simulink model "MHILSimHWImpl"  (R2024a)
settings: Solver=FixedStepDiscrete  StartTime=0.0  StopTime=2e-4  FixedStep=4e-9  RelTol=1e-3
values from neighbouring files (symbols this model uses):
  cfg = tddbl_model    [HILSimModel.m]
undefined symbols (not defined in the file or in its folder): AXI4, dt, hw, ip, Lite, xc7z020clg400
libraries: hdlBasic x1497, hdlUtilities x3, vmcUtilities x1
(part 2 of 11)

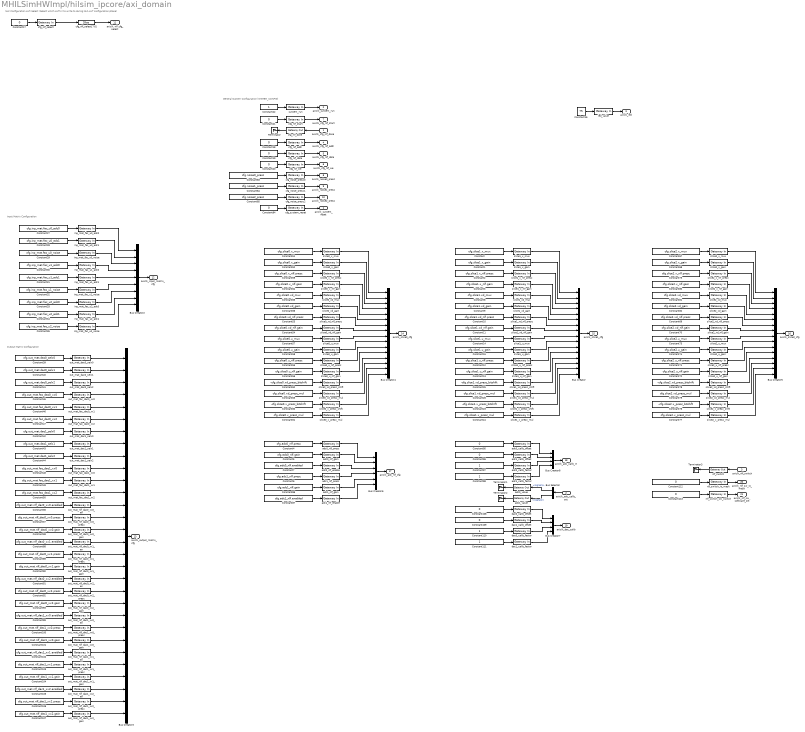
== system MHILSimHWImpl/hilsim_ipcore/axi_domain ==
  note: Input Matrix Configuration
  note: General System Configuration (SYSTEM_CONFIG)
  note: NLF Configuration LUT-Select (Select which LUT(s) to write to during NLF-LUT configuration phase)
  note: Output Matrix Configuration
  axiclk_cfg_nlf_done : Inport
  axiclk_adc_calib_out : Inport  Port=2
  axiclk_nlf_switch : Inport  Port=3
  Bus Creator : BusCreator  Inputs=16
  Bus Creator2 : BusCreator  Inputs=9
  Bus Creator3 : BusCreator  Inputs=30
  Bus Creator4 : BusCreator  Inputs=16
  Bus Creator5 : BusCreator  Inputs=16
  Bus Creator6 : BusCreator  Inputs=6
  Bus Creator7 : BusCreator  Inputs=4
  Bus Creator8 : BusCreator  Inputs=4
  Bus Selector : BusSelector  OutputSignals=signal1,signal2
  Constant : Constant  Value=cfg.slice1.x_mux
  Constant1 : Constant  Value=cfg.slice1.x_gain
  Constant10 : Constant  Value=cfg.slice1.xd_nlf.presc
  Constant100 : Constant  Value=cfg.out_mat.nlf_dac1_xx0.presc
  Constant101 : Constant  Value=cfg.out_mat.nlf_dac1_xx0.gain
  Constant102 : Constant  Value=cfg.out_mat.nlf_dac1_xx1.enabled
  Constant103 : Constant  Value=cfg.out_mat.nlf_dac1_xx1.presc
  Constant104 : Constant  Value=cfg.out_mat.nlf_dac1_xx1.gain
  Constant105 : Constant  Value=cfg.out_mat.nlf_dac1_xx2.enabled
  Constant106 : Constant  Value=cfg.out_mat.nlf_dac1_xx2.presc
  Constant107 : Constant  Value=cfg.out_mat.nlf_dac1_xx2.gain
  Constant{95,108,112..113} (4 alike) : Constant  Value=0  VectorParams1D=off
  Constant{17..21,94,96,109} (8 alike) : Constant  Value=0
  Constant11 : Constant  Value=cfg.slice1.xd_nlf.gain
  Constant{97..98,110..111} (4 alike) : Constant  VectorParams1D=off
  Constant12 : Constant  Value=cfg.slice1.u_nlf.presc
  Constant13 : Constant  Value=cfg.slice1.u_nlf.gain
  Constant14 : Constant  Value=cfg.slice1.u_mux
  Constant15 : Constant  Value=cfg.slice1.u_gain
  Constant16 : Constant  Value=75
  Constant2 : Constant  Value=cfg.slice1.x_nlf.presc
  Constant22 : Constant
  Constant23 : Constant  Value=-cfg.slice1.x_presc_bitshift  VectorParams1D=off
  Constant24 : Constant  Value=cfg.slice1.x_presc_mul
  Constant25 : Constant  Value=-cfg.slice1.xd_presc_bitshift
  Constant26 : Constant  Value=cfg.slice1.xd_presc_mul
  Constant27 : Constant  Value=cfg.inp_mat.fac_u0_adc0
  Constant28 : Constant  Value=cfg.inp_mat.fac_u0_adc1
  Constant29 : Constant  Value=cfg.inp_mat.fac_u0_noise
  Constant3 : Constant  Value=cfg.slice1.x_nlf.gain
  Constant30 : Constant  Value=cfg.inp_mat.fac_u1_adc0
  Constant31 : Constant  Value=cfg.inp_mat.fac_u1_adc1
  Constant32 : Constant  Value=cfg.inp_mat.fac_u1_noise
  Constant33 : Constant  Value=cfg.inp_mat.fac_u2_adc0
  Constant34 : Constant  Value=cfg.inp_mat.fac_u2_adc1
  Constant35 : Constant  Value=cfg.inp_mat.fac_u2_noise
  Constant36 : Constant  Value=cfg.out_mat.nlf_dac0_xx0.enabled
  Constant37 : Constant  Value=cfg.out_mat.nlf_dac0_xx0.presc
  Constant38 : Constant  Value=cfg.out_mat.nlf_dac0_xx0.gain
  Constant39 : Constant  Value=cfg.out_mat.dac0_selx0
  Constant4 : Constant  Value=cfg.adc0_nlf.presc
  Constant40 : Constant  Value=cfg.out_mat.dac0_selx1
  Constant41 : Constant  Value=cfg.out_mat.dac0_selx2
  Constant42 : Constant  Value=cfg.out_mat.dac1_selx0
  Constant43 : Constant  Value=cfg.out_mat.dac1_selx1
  Constant44 : Constant  Value=cfg.out_mat.dac1_selx2
  Constant45 : Constant  Value=cfg.out_mat.fac_dac0_xx0
  Constant46 : Constant  Value=cfg.out_mat.fac_dac0_xx1
  Constant47 : Constant  Value=cfg.out_mat.fac_dac0_xx2
  Constant48 : Constant  Value=cfg.out_mat.fac_dac1_xx0
  Constant49 : Constant  Value=cfg.out_mat.fac_dac1_xx1
  Constant5 : Constant  Value=cfg.adc0_nlf.gain
  Constant50 : Constant  Value=cfg.out_mat.fac_dac1_xx2
  Constant51 : Constant  Value=cfg.slice0.x_mux
  Constant52 : Constant  Value=cfg.slice0.x_gain
  Constant53 : Constant  Value=cfg.slice0.xd_nlf.presc
  Constant54 : Constant  Value=cfg.slice0.xd_nlf.gain
  Constant55 : Constant  Value=cfg.slice0.u_nlf.presc
  Constant56 : Constant  Value=cfg.slice0.u_nlf.gain
  Constant57 : Constant  Value=cfg.slice0.u_mux
  Constant58 : Constant  Value=cfg.slice0.u_gain
  Constant59 : Constant  Value=cfg.slice0.x_nlf.presc
  Constant6 : Constant  Value=cfg.adc1_nlf.presc
  Constant60 : Constant  Value=-cfg.slice0.x_presc_bitshift  VectorParams1D=off
  Constant61 : Constant  Value=cfg.slice0.x_presc_mul
  Constant62 : Constant  Value=-cfg.slice0.xd_presc_bitshift
  Constant63 : Constant  Value=cfg.slice0.xd_presc_mul
  Constant64 : Constant  Value=cfg.slice0.x_nlf.gain
  Constant65 : Constant  Value=cfg.slice0.xd_mux
  Constant66 : Constant  Value=cfg.slice0.xd_gain
  Constant67 : Constant  Value=cfg.slice2.x_mux
  Constant68 : Constant  Value=cfg.slice2.x_gain
  Constant69 : Constant  Value=cfg.slice2.xd_nlf.presc
  Constant7 : Constant  Value=cfg.adc0_nlf.enabled
  Constant70 : Constant  Value=cfg.slice2.xd_nlf.gain
  Constant71 : Constant  Value=cfg.slice2.u_nlf.presc
  Constant72 : Constant  Value=cfg.slice2.u_nlf.gain
  Constant73 : Constant  Value=cfg.slice2.u_mux
  Constant74 : Constant  Value=cfg.slice2.u_gain
  Constant75 : Constant  Value=cfg.slice2.x_nlf.presc
  Constant76 : Constant  Value=-cfg.slice2.x_presc_bitshift  VectorParams1D=off
  Constant77 : Constant  Value=cfg.slice2.x_presc_mul
  Constant78 : Constant  Value=-cfg.slice2.xd_presc_bitshift
  Constant79 : Constant  Value=cfg.slice2.xd_presc_mul
  Constant8 : Constant  Value=cfg.slice1.xd_mux
  Constant80 : Constant  Value=cfg.slice2.x_nlf.gain
  Constant81 : Constant  Value=cfg.slice2.xd_mux
  Constant82 : Constant  Value=cfg.slice2.xd_gain
  Constant83 : Constant  Value=cfg.noise0_presc
  Constant84 : Constant  Value=cfg.noise1_presc
  Constant85 : Constant  Value=cfg.noise2_presc
  Constant86 : Constant  Value=cfg.adc1_nlf.gain
  Constant87 : Constant  Value=cfg.adc1_nlf.enabled
  Constant88 : Constant  Value=cfg.out_mat.nlf_dac0_xx1.enabled
  Constant89 : Constant  Value=cfg.out_mat.nlf_dac0_xx1.presc
  Constant9 : Constant  Value=cfg.slice1.xd_gain
  Constant90 : Constant  Value=cfg.out_mat.nlf_dac0_xx1.gain
  Constant91 : Constant  Value=cfg.out_mat.nlf_dac0_xx2.enabled
  Constant92 : Constant  Value=cfg.out_mat.nlf_dac0_xx2.presc
  Constant93 : Constant  Value=cfg.out_mat.nlf_dac0_xx2.gain
  Constant99 : Constant  Value=cfg.out_mat.nlf_dac1_xx0.enabled
  Terminator{,1..3} (4 alike) : Terminator
  adc0_calib_factor : hdlBasic/Gateway In  gui_display_data_type=Fixed-point  arith_type=Signed (2's comp)  n_bits=dt.const.sz  bin_pt=dt.const.bin  preci_type=Single  exp_width=8  frac_width=24  rows=1  columns=1  quantization=Truncate  overflow=Wrap  period=hw.t_axi  UseAsADC=off  ADCChannel='1'  interface=AXI4-Lite  automatic_assignment=off  address_offset=ip.offsets.calib + hex2dec('08')  intf_name='axi_b'  intf_description=''  default_value=0  timing_constraint=None  locs_specified=off  LOCs={}  io_standard={}  inherit_from_input=off  hdl_port=on  XmcBlockStatus=1  maskContainerNames=group4  block_type=gatewayin  block_config=sysgen:gateway_in_config  block_width_w=590  block_height_w=620  block_width=640  block_height=850
  adc0_calib_offset : hdlBasic/Gateway In  gui_display_data_type=Fixed-point  arith_type=Signed (2's comp)  n_bits=dt.slice.sz  bin_pt=dt.slice.bin  preci_type=Single  exp_width=8  frac_width=24  rows=1  columns=1  quantization=Truncate  overflow=Wrap  period=hw.t_axi  UseAsADC=off  ADCChannel='1'  interface=AXI4-Lite  automatic_assignment=off  address_offset=ip.offsets.calib + hex2dec('00')  intf_name='axi_b'  intf_description=''  default_value=0  timing_constraint=None  locs_specified=off  LOCs={}  io_standard={}  inherit_from_input=off  hdl_port=on  XmcBlockStatus=1  maskContainerNames=group4  block_type=gatewayin  block_config=sysgen:gateway_in_config  block_width_w=590  block_height_w=620  block_width=640  block_height=850
  adc0_nlf_enable : hdlBasic/Gateway In  gui_display_data_type=Boolean  arith_type=Boolean  n_bits=8  bin_pt=0  preci_type=Single  exp_width=8  frac_width=24  rows=1  columns=1  quantization=Truncate  overflow=Wrap  period=hw.t_axi  UseAsADC=off  ADCChannel='1'  interface=AXI4-Lite  automatic_assignment=off  address_offset=ip.offsets.adc_nlf_cfg + hex2dec('08')  intf_name=''  intf_description=''  default_value=0  timing_constraint=None  locs_specified=off  LOCs={}  io_standard={}  inherit_from_input=off  hdl_port=on  XmcBlockStatus=1  maskContainerNames=group4  block_type=gatewayin  block_config=sysgen:gateway_in_config  block_width_w=590  block_height_w=620  block_width=640  block_height=850
  adc0_nlf_gain : hdlBasic/Gateway In  gui_display_data_type=Fixed-point  arith_type=Signed (2's comp)  n_bits=dt.const.sz  bin_pt=dt.const.bin  preci_type=Single  exp_width=8  frac_width=24  rows=1  columns=1  quantization=Truncate  overflow=Wrap  period=hw.t_axi  UseAsADC=off  ADCChannel='1'  interface=AXI4-Lite  automatic_assignment=off  address_offset=ip.offsets.adc_nlf_cfg + hex2dec('04')  intf_name=''  intf_description=''  default_value=0  timing_constraint=None  locs_specified=off  LOCs={}  io_standard={}  inherit_from_input=off  hdl_port=on  XmcBlockStatus=1  maskContainerNames=group4  block_type=gatewayin  block_config=sysgen:gateway_in_config  block_width_w=590  block_height_w=620  block_width=640  block_height=850
  adc0_nlf_presc : hdlBasic/Gateway In  gui_display_data_type=Fixed-point  arith_type=Signed (2's comp)  n_bits=dt.const.sz  bin_pt=dt.const.bin  preci_type=Single  exp_width=8  frac_width=24  rows=1  columns=1  quantization=Truncate  overflow=Wrap  period=hw.t_axi  UseAsADC=off  ADCChannel='1'  interface=AXI4-Lite  automatic_assignment=off  address_offset=ip.offsets.adc_nlf_cfg + hex2dec('00')  intf_name=''  intf_description=''  default_value=0  timing_constraint=None  locs_specified=off  LOCs={}  io_standard={}  inherit_from_input=off  hdl_port=on  XmcBlockStatus=1  maskContainerNames=group4  block_type=gatewayin  block_config=sysgen:gateway_in_config  block_width_w=590  block_height_w=620  block_width=640  block_height=850
  adc0_value : hdlBasic/Gateway Out  inherit_from_input=off  hdl_port=on  rows=1  columns=1  UseAsDAC=off  DACChannel='1'  interface=AXI4-Lite  automatic_assignment=off  address_offset=ip.offsets.calib + hex2dec('10')  intf_name='axi_b'  intf_description=''  timing_constraint=None  locs_specified=off  LOCs={}  io_standard={}  XmcBlockStatus=1  maskContainerNames=group4  block_type=gatewayout  block_config=sysgen:gateway_out_config  block_width_w=590  block_height_w=620  block_width=620  block_height=750
  adc1_calib_factor : hdlBasic/Gateway In  gui_display_data_type=Fixed-point  arith_type=Signed (2's comp)  n_bits=dt.const.sz  bin_pt=dt.const.bin  preci_type=Single  exp_width=8  frac_width=24  rows=1  columns=1  quantization=Truncate  overflow=Wrap  period=hw.t_axi  UseAsADC=off  ADCChannel='1'  interface=AXI4-Lite  automatic_assignment=off  address_offset=ip.offsets.calib + hex2dec('0c')  intf_name='axi_b'  intf_description=''  default_value=0  timing_constraint=None  locs_specified=off  LOCs={}  io_standard={}  inherit_from_input=off  hdl_port=on  XmcBlockStatus=1  maskContainerNames=group4  block_type=gatewayin  block_config=sysgen:gateway_in_config  block_width_w=590  block_height_w=620  block_width=640  block_height=850
  adc1_calib_offset : hdlBasic/Gateway In  gui_display_data_type=Fixed-point  arith_type=Signed (2's comp)  n_bits=dt.slice.sz  bin_pt=dt.slice.bin  preci_type=Single  exp_width=8  frac_width=24  rows=1  columns=1  quantization=Truncate  overflow=Wrap  period=hw.t_axi  UseAsADC=off  ADCChannel='1'  interface=AXI4-Lite  automatic_assignment=off  address_offset=ip.offsets.calib + hex2dec('04')  intf_name='axi_b'  intf_description=''  default_value=0  timing_constraint=None  locs_specified=off  LOCs={}  io_standard={}  inherit_from_input=off  hdl_port=on  XmcBlockStatus=1  maskContainerNames=group4  block_type=gatewayin  block_config=sysgen:gateway_in_config  block_width_w=590  block_height_w=620  block_width=640  block_height=850
  adc1_nlf_enable : hdlBasic/Gateway In  gui_display_data_type=Boolean  arith_type=Boolean  n_bits=8  bin_pt=0  preci_type=Single  exp_width=8  frac_width=24  rows=1  columns=1  quantization=Truncate  overflow=Wrap  period=hw.t_axi  UseAsADC=off  ADCChannel='1'  interface=AXI4-Lite  automatic_assignment=off  address_offset=ip.offsets.adc_nlf_cfg + hex2dec('14')  intf_name=''  intf_description=''  default_value=0  timing_constraint=None  locs_specified=off  LOCs={}  io_standard={}  inherit_from_input=off  hdl_port=on  XmcBlockStatus=1  maskContainerNames=group4  block_type=gatewayin  block_config=sysgen:gateway_in_config  block_width_w=590  block_height_w=620  block_width=640  block_height=850
  adc1_nlf_gain : hdlBasic/Gateway In  gui_display_data_type=Fixed-point  arith_type=Signed (2's comp)  n_bits=dt.const.sz  bin_pt=dt.const.bin  preci_type=Single  exp_width=8  frac_width=24  rows=1  columns=1  quantization=Truncate  overflow=Wrap  period=hw.t_axi  UseAsADC=off  ADCChannel='1'  interface=AXI4-Lite  automatic_assignment=off  address_offset=ip.offsets.adc_nlf_cfg + hex2dec('10')  intf_name=''  intf_description=''  default_value=0  timing_constraint=None  locs_specified=off  LOCs={}  io_standard={}  inherit_from_input=off  hdl_port=on  XmcBlockStatus=1  maskContainerNames=group4  block_type=gatewayin  block_config=sysgen:gateway_in_config  block_width_w=590  block_height_w=620  block_width=640  block_height=850
  adc1_nlf_presc : hdlBasic/Gateway In  gui_display_data_type=Fixed-point  arith_type=Signed (2's comp)  n_bits=dt.const.sz  bin_pt=dt.const.bin  preci_type=Single  exp_width=8  frac_width=24  rows=1  columns=1  quantization=Truncate  overflow=Wrap  period=hw.t_axi  UseAsADC=off  ADCChannel='1'  interface=AXI4-Lite  automatic_assignment=off  address_offset=ip.offsets.adc_nlf_cfg + hex2dec('0c')  intf_name=''  intf_description=''  default_value=0  timing_constraint=None  locs_specified=off  LOCs={}  io_standard={}  inherit_from_input=off  hdl_port=on  XmcBlockStatus=1  maskContainerNames=group4  block_type=gatewayin  block_config=sysgen:gateway_in_config  block_width_w=590  block_height_w=620  block_width=640  block_height=850
  adc1_value : hdlBasic/Gateway Out  inherit_from_input=off  hdl_port=on  rows=1  columns=1  UseAsDAC=off  DACChannel='1'  interface=AXI4-Lite  automatic_assignment=off  address_offset=ip.offsets.calib + hex2dec('14')  intf_name='axi_b'  intf_description=''  timing_constraint=None  locs_specified=off  LOCs={}  io_standard={}  XmcBlockStatus=1  maskContainerNames=group4  block_type=gatewayout  block_config=sysgen:gateway_out_config  block_width_w=590  block_height_w=620  block_width=620  block_height=750
  cfg_nlf_addr : hdlBasic/Gateway In  gui_display_data_type=Fixed-point  arith_type=Unsigned  n_bits=ip.f_nlf.lut_addr_bits  bin_pt=0  preci_type=Single  exp_width=8  frac_width=24  rows=1  columns=1  quantization=Truncate  overflow=Wrap  period=hw.t_axi  UseAsADC=off  ADCChannel='1'  interface=AXI4-Lite  automatic_assignment=off  address_offset=ip.offsets.system_cfg + hex2dec('14')  intf_name=''  intf_description=''  default_value=0  timing_constraint=None  locs_specified=off  LOCs={}  io_standard={}  inherit_from_input=off  hdl_port=on  XmcBlockStatus=1  maskContainerNames=group4  block_type=gatewayin  block_config=sysgen:gateway_in_config  block_width_w=590  block_height_w=620  block_width=640  block_height=850
  cfg_nlf_data : hdlBasic/Gateway In  gui_display_data_type=Fixed-point  arith_type=Signed (2's comp)  n_bits=dt.nlf.sz  bin_pt=dt.nlf.bin  preci_type=Single  exp_width=8  frac_width=24  rows=1  columns=1  quantization=Truncate  overflow=Wrap  period=hw.t_axi  UseAsADC=off  ADCChannel='1'  interface=AXI4-Lite  automatic_assignment=off  address_offset=ip.offsets.system_cfg + hex2dec('18')  intf_name=''  intf_description=''  default_value=0  timing_constraint=None  locs_specified=off  LOCs={}  io_standard={}  inherit_from_input=off  hdl_port=on  XmcBlockStatus=1  maskContainerNames=group4  block_type=gatewayin  block_config=sysgen:gateway_in_config  block_width_w=590  block_height_w=620  block_width=640  block_height=850
  cfg_nlf_done : hdlBasic/Gateway Out  inherit_from_input=off  hdl_port=on  rows=1  columns=1  UseAsDAC=off  DACChannel='1'  interface=AXI4-Lite  automatic_assignment=off  address_offset=ip.offsets.system_cfg + hex2dec('08')  intf_name=''  intf_description=''  timing_constraint=None  locs_specified=off  LOCs={}  io_standard={}  XmcBlockStatus=1  maskContainerNames=group4  block_type=gatewayout  block_config=sysgen:gateway_out_config  block_width_w=590  block_height_w=620  block_width=620  block_height=750
  cfg_nlf_select : hdlBasic/Gateway In  gui_display_data_type=Fixed-point  arith_type=Unsigned  n_bits=32  bin_pt=0  preci_type=Single  exp_width=8  frac_width=24  rows=1  columns=1  quantization=Truncate  overflow=Wrap  period=hw.t_axi  UseAsADC=off  ADCChannel='1'  interface=AXI4-Lite  automatic_assignment=off  address_offset=ip.offsets.system_cfg + hex2dec('10')  intf_name=''  intf_description=''  default_value=0  timing_constraint=None  locs_specified=off  LOCs={}  io_standard={}  inherit_from_input=off  hdl_port=on  XmcBlockStatus=1  maskContainerNames=group4  block_type=gatewayin  block_config=sysgen:gateway_in_config  block_width_w=590  block_height_w=620  block_width=640  block_height=850
  cfg_nlf_select[7:0] : hdlBasic/Slice  nbits=8  boolean_output=off  mode=Lower Bit Location + Width  bit1=0  base1=MSB of Input  bit0=0  base0=LSB of Input  XmcBlockStatus=1  maskContainerNames=group1  block_type=slice  block_config=sysgen:Slice_config
  cfg_nlf_start : hdlBasic/Gateway In  gui_display_data_type=Boolean  arith_type=Boolean  n_bits=dt.nlf.sz  bin_pt=dt.nlf.bin  preci_type=Single  exp_width=8  frac_width=24  rows=1  columns=1  quantization=Truncate  overflow=Wrap  period=hw.t_axi  UseAsADC=off  ADCChannel='1'  interface=AXI4-Lite  automatic_assignment=off  address_offset=ip.offsets.system_cfg + hex2dec('04')  intf_name=''  intf_description=''  default_value=0  timing_constraint=None  locs_specified=off  LOCs={}  io_standard={}  inherit_from_input=off  hdl_port=on  XmcBlockStatus=1  maskContainerNames=group4  block_type=gatewayin  block_config=sysgen:gateway_in_config  block_width_w=590  block_height_w=620  block_width=640  block_height=850
  cfg_nlf_we : hdlBasic/Gateway In  gui_display_data_type=Boolean  arith_type=Boolean  n_bits=dt.nlf.sz  bin_pt=dt.nlf.bin  preci_type=Single  exp_width=8  frac_width=24  rows=1  columns=1  quantization=Truncate  overflow=Wrap  period=hw.t_axi  UseAsADC=off  ADCChannel='1'  interface=AXI4-Lite  automatic_assignment=off  address_offset=ip.offsets.system_cfg + hex2dec('0c')  intf_name=''  intf_description=''  default_value=0  timing_constraint=None  locs_specified=off  LOCs={}  io_standard={}  inherit_from_input=off  hdl_port=on  XmcBlockStatus=1  maskContainerNames=group4  block_type=gatewayin  block_config=sysgen:gateway_in_config  block_width_w=590  block_height_w=620  block_width=640  block_height=850
  cfg_noise_presc0 : hdlBasic/Gateway In  gui_display_data_type=Fixed-point  arith_type=Signed (2's comp)  n_bits=dt.const.sz  bin_pt=dt.const.bin  preci_type=Single  exp_width=8  frac_width=24  rows=1  columns=1  quantization=Truncate  overflow=Wrap  period=hw.t_axi  UseAsADC=off  ADCChannel='1'  interface=AXI4-Lite  automatic_assignment=off  address_offset=ip.offsets.system_cfg + hex2dec('1c')  intf_name=''  intf_description=''  default_value=0  timing_constraint=None  locs_specified=off  LOCs={}  io_standard={}  inherit_from_input=off  hdl_port=on  XmcBlockStatus=1  maskContainerNames=group4  block_type=gatewayin  block_config=sysgen:gateway_in_config  block_width_w=590  block_height_w=620  block_width=640  block_height=850
  cfg_noise_presc1 : hdlBasic/Gateway In  gui_display_data_type=Fixed-point  arith_type=Signed (2's comp)  n_bits=dt.const.sz  bin_pt=dt.const.bin  preci_type=Single  exp_width=8  frac_width=24  rows=1  columns=1  quantization=Truncate  overflow=Wrap  period=hw.t_axi  UseAsADC=off  ADCChannel='1'  interface=AXI4-Lite  automatic_assignment=off  address_offset=ip.offsets.system_cfg + hex2dec('20')  intf_name=''  intf_description=''  default_value=0  timing_constraint=None  locs_specified=off  LOCs={}  io_standard={}  inherit_from_input=off  hdl_port=on  XmcBlockStatus=1  maskContainerNames=group4  block_type=gatewayin  block_config=sysgen:gateway_in_config  block_width_w=590  block_height_w=620  block_width=640  block_height=850
  cfg_noise_presc2 : hdlBasic/Gateway In  gui_display_data_type=Fixed-point  arith_type=Signed (2's comp)  n_bits=dt.const.sz  bin_pt=dt.const.bin  preci_type=Single  exp_width=8  frac_width=24  rows=1  columns=1  quantization=Truncate  overflow=Wrap  period=hw.t_axi  UseAsADC=off  ADCChannel='1'  interface=AXI4-Lite  automatic_assignment=off  address_offset=ip.offsets.system_cfg + hex2dec('24')  intf_name=''  intf_description=''  default_value=0  timing_constraint=None  locs_specified=off  LOCs={}  io_standard={}  inherit_from_input=off  hdl_port=on  XmcBlockStatus=1  maskContainerNames=group4  block_type=gatewayin  block_config=sysgen:gateway_in_config  block_width_w=590  block_height_w=620  block_width=640  block_height=850
  cfg_system_reset : hdlBasic/Gateway In  gui_display_data_type=Boolean  arith_type=Boolean  n_bits=dt.const.sz  bin_pt=dt.const.bin  preci_type=Single  exp_width=8  frac_width=24  rows=1  columns=1  quantization=Truncate  overflow=Wrap  period=hw.t_axi  UseAsADC=off  ADCChannel='1'  interface=AXI4-Lite  automatic_assignment=off  address_offset=ip.offsets.system_cfg + hex2dec('28')  intf_name=''  intf_description=''  default_value=0  timing_constraint=None  locs_specified=off  LOCs={}  io_standard={}  inherit_from_input=off  hdl_port=on  XmcBlockStatus=1  maskContainerNames=group4  block_type=gatewayin  block_config=sysgen:gateway_in_config  block_width_w=590  block_height_w=620  block_width=640  block_height=850
  dac0_calib_factor : hdlBasic/Gateway In  gui_display_data_type=Fixed-point  arith_type=Signed (2's comp)  n_bits=dt.const.sz  bin_pt=dt.const.bin  preci_type=Single  exp_width=8  frac_width=24  rows=1  columns=1  quantization=Truncate  overflow=Wrap  period=hw.t_axi  UseAsADC=off  ADCChannel='1'  interface=AXI4-Lite  automatic_assignment=off  address_offset=ip.offsets.calib + hex2dec('20')  intf_name='axi_b'  intf_description=''  default_value=0  timing_constraint=None  locs_specified=off  LOCs={}  io_standard={}  inherit_from_input=off  hdl_port=on  XmcBlockStatus=1  maskContainerNames=group4  block_type=gatewayin  block_config=sysgen:gateway_in_config  block_width_w=590  block_height_w=620  block_width=640  block_height=850
  dac0_calib_offset : hdlBasic/Gateway In  gui_display_data_type=Fixed-point  arith_type=Signed (2's comp)  n_bits=dt.slice.sz  bin_pt=dt.slice.bin  preci_type=Single  exp_width=8  frac_width=24  rows=1  columns=1  quantization=Truncate  overflow=Wrap  period=hw.t_axi  UseAsADC=off  ADCChannel='1'  interface=AXI4-Lite  automatic_assignment=off  address_offset=ip.offsets.calib + hex2dec('18')  intf_name='axi_b'  intf_description=''  default_value=0  timing_constraint=None  locs_specified=off  LOCs={}  io_standard={}  inherit_from_input=off  hdl_port=on  XmcBlockStatus=1  maskContainerNames=group4  block_type=gatewayin  block_config=sysgen:gateway_in_config  block_width_w=590  block_height_w=620  block_width=640  block_height=850
  dac1_calib_factor : hdlBasic/Gateway In  gui_display_data_type=Fixed-point  arith_type=Signed (2's comp)  n_bits=dt.const.sz  bin_pt=dt.const.bin  preci_type=Single  exp_width=8  frac_width=24  rows=1  columns=1  quantization=Truncate  overflow=Wrap  period=hw.t_axi  UseAsADC=off  ADCChannel='1'  interface=AXI4-Lite  automatic_assignment=off  address_offset=ip.offsets.calib + hex2dec('24')  intf_name='axi_b'  intf_description=''  default_value=0  timing_constraint=None  locs_specified=off  LOCs={}  io_standard={}  inherit_from_input=off  hdl_port=on  XmcBlockStatus=1  maskContainerNames=group4  block_type=gatewayin  block_config=sysgen:gateway_in_config  block_width_w=590  block_height_w=620  block_width=640  block_height=850
  dac1_calib_offset : hdlBasic/Gateway In  gui_display_data_type=Fixed-point  arith_type=Signed (2's comp)  n_bits=dt.slice.sz  bin_pt=dt.slice.bin  preci_type=Single  exp_width=8  frac_width=24  rows=1  columns=1  quantization=Truncate  overflow=Wrap  period=hw.t_axi  UseAsADC=off  ADCChannel='1'  interface=AXI4-Lite  automatic_assignment=off  address_offset=ip.offsets.calib + hex2dec('1c')  intf_name='axi_b'  intf_description=''  default_value=0  timing_constraint=None  locs_specified=off  LOCs={}  io_standard={}  inherit_from_input=off  hdl_port=on  XmcBlockStatus=1  maskContainerNames=group4  block_type=gatewayin  block_config=sysgen:gateway_in_config  block_width_w=590  block_height_w=620  block_width=640  block_height=850
  inp_mat_fac_u0_adc0 : hdlBasic/Gateway In  gui_display_data_type=Fixed-point  arith_type=Signed (2's comp)  n_bits=dt.const.sz  bin_pt=dt.const.bin  preci_type=Single  exp_width=8  frac_width=24  rows=1  columns=1  quantization=Truncate  overflow=Wrap  period=hw.t_axi  UseAsADC=off  ADCChannel='1'  interface=AXI4-Lite  automatic_assignment=off  address_offset=ip.offsets.input_mat_cfg + hex2dec('00')  intf_name=''  intf_description=''  default_value=0  timing_constraint=None  locs_specified=off  LOCs={}  io_standard={}  inherit_from_input=off  hdl_port=on  XmcBlockStatus=1  maskContainerNames=group4  block_type=gatewayin  block_config=sysgen:gateway_in_config  block_width_w=590  block_height_w=620  block_width=640  block_height=850
  inp_mat_fac_u0_adc1 : hdlBasic/Gateway In  gui_display_data_type=Fixed-point  arith_type=Signed (2's comp)  n_bits=dt.const.sz  bin_pt=dt.const.bin  preci_type=Single  exp_width=8  frac_width=24  rows=1  columns=1  quantization=Truncate  overflow=Wrap  period=hw.t_axi  UseAsADC=off  ADCChannel='1'  interface=AXI4-Lite  automatic_assignment=off  address_offset=ip.offsets.input_mat_cfg + hex2dec('04')  intf_name=''  intf_description=''  default_value=0  timing_constraint=None  locs_specified=off  LOCs={}  io_standard={}  inherit_from_input=off  hdl_port=on  XmcBlockStatus=1  maskContainerNames=group4  block_type=gatewayin  block_config=sysgen:gateway_in_config  block_width_w=590  block_height_w=620  block_width=640  block_height=850
  inp_mat_fac_u0_noise : hdlBasic/Gateway In  gui_display_data_type=Fixed-point  arith_type=Signed (2's comp)  n_bits=dt.const.sz  bin_pt=dt.const.bin  preci_type=Single  exp_width=8  frac_width=24  rows=1  columns=1  quantization=Truncate  overflow=Wrap  period=hw.t_axi  UseAsADC=off  ADCChannel='1'  interface=AXI4-Lite  automatic_assignment=off  address_offset=ip.offsets.input_mat_cfg + hex2dec('08')  intf_name=''  intf_description=''  default_value=0  timing_constraint=None  locs_specified=off  LOCs={}  io_standard={}  inherit_from_input=off  hdl_port=on  XmcBlockStatus=1  maskContainerNames=group4  block_type=gatewayin  block_config=sysgen:gateway_in_config  block_width_w=590  block_height_w=620  block_width=640  block_height=850
  inp_mat_fac_u1_adc0 : hdlBasic/Gateway In  gui_display_data_type=Fixed-point  arith_type=Signed (2's comp)  n_bits=dt.const.sz  bin_pt=dt.const.bin  preci_type=Single  exp_width=8  frac_width=24  rows=1  columns=1  quantization=Truncate  overflow=Wrap  period=hw.t_axi  UseAsADC=off  ADCChannel='1'  interface=AXI4-Lite  automatic_assignment=off  address_offset=ip.offsets.input_mat_cfg + hex2dec('0c')  intf_name=''  intf_description=''  default_value=0  timing_constraint=None  locs_specified=off  LOCs={}  io_standard={}  inherit_from_input=off  hdl_port=on  XmcBlockStatus=1  maskContainerNames=group4  block_type=gatewayin  block_config=sysgen:gateway_in_config  block_width_w=590  block_height_w=620  block_width=640  block_height=850
  inp_mat_fac_u1_adc1 : hdlBasic/Gateway In  gui_display_data_type=Fixed-point  arith_type=Signed (2's comp)  n_bits=dt.const.sz  bin_pt=dt.const.bin  preci_type=Single  exp_width=8  frac_width=24  rows=1  columns=1  quantization=Truncate  overflow=Wrap  period=hw.t_axi  UseAsADC=off  ADCChannel='1'  interface=AXI4-Lite  automatic_assignment=off  address_offset=ip.offsets.input_mat_cfg + hex2dec('10')  intf_name=''  intf_description=''  default_value=0  timing_constraint=None  locs_specified=off  LOCs={}  io_standard={}  inherit_from_input=off  hdl_port=on  XmcBlockStatus=1  maskContainerNames=group4  block_type=gatewayin  block_config=sysgen:gateway_in_config  block_width_w=590  block_height_w=620  block_width=640  block_height=850
  inp_mat_fac_u1_noise : hdlBasic/Gateway In  gui_display_data_type=Fixed-point  arith_type=Signed (2's comp)  n_bits=dt.const.sz  bin_pt=dt.const.bin  preci_type=Single  exp_width=8  frac_width=24  rows=1  columns=1  quantization=Truncate  overflow=Wrap  period=hw.t_axi  UseAsADC=off  ADCChannel='1'  interface=AXI4-Lite  automatic_assignment=off  address_offset=ip.offsets.input_mat_cfg + hex2dec('14')  intf_name=''  intf_description=''  default_value=0  timing_constraint=None  locs_specified=off  LOCs={}  io_standard={}  inherit_from_input=off  hdl_port=on  XmcBlockStatus=1  maskContainerNames=group4  block_type=gatewayin  block_config=sysgen:gateway_in_config  block_width_w=590  block_height_w=620  block_width=640  block_height=850
  inp_mat_fac_u2_adc0 : hdlBasic/Gateway In  gui_display_data_type=Fixed-point  arith_type=Signed (2's comp)  n_bits=dt.const.sz  bin_pt=dt.const.bin  preci_type=Single  exp_width=8  frac_width=24  rows=1  columns=1  quantization=Truncate  overflow=Wrap  period=hw.t_axi  UseAsADC=off  ADCChannel='1'  interface=AXI4-Lite  automatic_assignment=off  address_offset=ip.offsets.input_mat_cfg + hex2dec('18')  intf_name=''  intf_description=''  default_value=0  timing_constraint=None  locs_specified=off  LOCs={}  io_standard={}  inherit_from_input=off  hdl_port=on  XmcBlockStatus=1  maskContainerNames=group4  block_type=gatewayin  block_config=sysgen:gateway_in_config  block_width_w=590  block_height_w=620  block_width=640  block_height=850
  inp_mat_fac_u2_adc1 : hdlBasic/Gateway In  gui_display_data_type=Fixed-point  arith_type=Signed (2's comp)  n_bits=dt.const.sz  bin_pt=dt.const.bin  preci_type=Single  exp_width=8  frac_width=24  rows=1  columns=1  quantization=Truncate  overflow=Wrap  period=hw.t_axi  UseAsADC=off  ADCChannel='1'  interface=AXI4-Lite  automatic_assignment=off  address_offset=ip.offsets.input_mat_cfg + hex2dec('1c')  intf_name=''  intf_description=''  default_value=0  timing_constraint=None  locs_specified=off  LOCs={}  io_standard={}  inherit_from_input=off  hdl_port=on  XmcBlockStatus=1  maskContainerNames=group4  block_type=gatewayin  block_config=sysgen:gateway_in_config  block_width_w=590  block_height_w=620  block_width=640  block_height=850
  inp_mat_fac_u2_noise : hdlBasic/Gateway In  gui_display_data_type=Fixed-point  arith_type=Signed (2's comp)  n_bits=dt.const.sz  bin_pt=dt.const.bin  preci_type=Single  exp_width=8  frac_width=24  rows=1  columns=1  quantization=Truncate  overflow=Wrap  period=hw.t_axi  UseAsADC=off  ADCChannel='1'  interface=AXI4-Lite  automatic_assignment=off  address_offset=ip.offsets.input_mat_cfg + hex2dec('20')  intf_name=''  intf_description=''  default_value=0  timing_constraint=None  locs_specified=off  LOCs={}  io_standard={}  inherit_from_input=off  hdl_port=on  XmcBlockStatus=1  maskContainerNames=group4  block_type=gatewayin  block_config=sysgen:gateway_in_config  block_width_w=590  block_height_w=620  block_width=640  block_height=850
  led_value : hdlBasic/Gateway In  gui_display_data_type=Fixed-point  arith_type=Unsigned  n_bits=8  bin_pt=0  preci_type=Single  exp_width=8  frac_width=24  rows=1  columns=1  quantization=Truncate  overflow=Wrap  period=hw.t_axi  UseAsADC=off  ADCChannel='1'  interface=AXI4-Lite  automatic_assignment=off  address_offset=ip.offsets.led  intf_name=''  intf_description=''  default_value=0  timing_constraint=None  locs_specified=off  LOCs={}  io_standard={}  inherit_from_input=off  hdl_port=on  XmcBlockStatus=1  maskContainerNames=group4  block_type=gatewayin  block_config=sysgen:gateway_in_config  block_width_w=590  block_height_w=620  block_width=640  block_height=850
  nlf_switch : hdlBasic/Gateway Out  inherit_from_input=off  hdl_port=on  rows=1  columns=1  UseAsDAC=off  DACChannel='1'  interface=AXI4-Lite  automatic_assignment=off  address_offset=ip.offsets.nlf_switch + hex2dec('00')  intf_name='axi_b'  intf_description=''  timing_constraint=None  locs_specified=off  LOCs={}  io_standard={}  XmcBlockStatus=1  maskContainerNames=group4  block_type=gatewayout  block_config=sysgen:gateway_out_config  block_width_w=590  block_height_w=620  block_width=620  block_height=750
  nlf_switch_io_mask : hdlBasic/Gateway In  gui_display_data_type=Fixed-point  arith_type=Unsigned  n_bits=9  bin_pt=0  preci_type=Single  exp_width=8  frac_width=24  rows=1  columns=1  quantization=Truncate  overflow=Wrap  period=hw.t_axi  UseAsADC=off  ADCChannel='1'  interface=AXI4-Lite  automatic_assignment=off  address_offset=ip.offsets.nlf_switch + hex2dec('04')  intf_name='axi_b'  intf_description=''  default_value=0  timing_constraint=None  locs_specified=off  LOCs={}  io_standard={}  inherit_from_input=off  hdl_port=on  XmcBlockStatus=1  maskContainerNames=group4  block_type=gatewayin  block_config=sysgen:gateway_in_config  block_width_w=590  block_height_w=620  block_width=640  block_height=850
  nlf_switch_sw_switch : hdlBasic/Gateway In  gui_display_data_type=Fixed-point  arith_type=Unsigned  n_bits=9  bin_pt=0  preci_type=Single  exp_width=8  frac_width=24  rows=1  columns=1  quantization=Truncate  overflow=Wrap  period=hw.t_axi  UseAsADC=off  ADCChannel='1'  interface=AXI4-Lite  automatic_assignment=off  address_offset=ip.offsets.nlf_switch + hex2dec('08')  intf_name='axi_b'  intf_description=''  default_value=0  timing_constraint=None  locs_specified=off  LOCs={}  io_standard={}  inherit_from_input=off  hdl_port=on  XmcBlockStatus=1  maskContainerNames=group4  block_type=gatewayin  block_config=sysgen:gateway_in_config  block_width_w=590  block_height_w=620  block_width=640  block_height=850
  out_mat_dac0_selx0 : hdlBasic/Gateway In  gui_display_data_type=Fixed-point  arith_type=Unsigned  n_bits=2  bin_pt=0  preci_type=Single  exp_width=8  frac_width=24  rows=1  columns=1  quantization=Truncate  overflow=Wrap  period=hw.t_axi  UseAsADC=off  ADCChannel='1'  interface=AXI4-Lite  automatic_assignment=off  address_offset=ip.offsets.output_mat_cfg + hex2dec('00')  intf_name=''  intf_description=''  default_value=0  timing_constraint=None  locs_specified=off  LOCs={}  io_standard={}  inherit_from_input=off  hdl_port=on  XmcBlockStatus=1  maskContainerNames=group4  block_type=gatewayin  block_config=sysgen:gateway_in_config  block_width_w=590  block_height_w=620  block_width=640  block_height=850
  out_mat_dac0_selx1 : hdlBasic/Gateway In  gui_display_data_type=Fixed-point  arith_type=Unsigned  n_bits=2  bin_pt=0  preci_type=Single  exp_width=8  frac_width=24  rows=1  columns=1  quantization=Truncate  overflow=Wrap  period=hw.t_axi  UseAsADC=off  ADCChannel='1'  interface=AXI4-Lite  automatic_assignment=off  address_offset=ip.offsets.output_mat_cfg + hex2dec('04')  intf_name=''  intf_description=''  default_value=0  timing_constraint=None  locs_specified=off  LOCs={}  io_standard={}  inherit_from_input=off  hdl_port=on  XmcBlockStatus=1  maskContainerNames=group4  block_type=gatewayin  block_config=sysgen:gateway_in_config  block_width_w=590  block_height_w=620  block_width=640  block_height=850
  out_mat_dac0_selx2 : hdlBasic/Gateway In  gui_display_data_type=Fixed-point  arith_type=Unsigned  n_bits=2  bin_pt=0  preci_type=Single  exp_width=8  frac_width=24  rows=1  columns=1  quantization=Truncate  overflow=Wrap  period=hw.t_axi  UseAsADC=off  ADCChannel='1'  interface=AXI4-Lite  automatic_assignment=off  address_offset=ip.offsets.output_mat_cfg + hex2dec('08')  intf_name=''  intf_description=''  default_value=0  timing_constraint=None  locs_specified=off  LOCs={}  io_standard={}  inherit_from_input=off  hdl_port=on  XmcBlockStatus=1  maskContainerNames=group4  block_type=gatewayin  block_config=sysgen:gateway_in_config  block_width_w=590  block_height_w=620  block_width=640  block_height=850
  out_mat_dac1_selx0 : hdlBasic/Gateway In  gui_display_data_type=Fixed-point  arith_type=Unsigned  n_bits=2  bin_pt=0  preci_type=Single  exp_width=8  frac_width=24  rows=1  columns=1  quantization=Truncate  overflow=Wrap  period=hw.t_axi  UseAsADC=off  ADCChannel='1'  interface=AXI4-Lite  automatic_assignment=off  address_offset=ip.offsets.output_mat_cfg + hex2dec('18')  intf_name=''  intf_description=''  default_value=0  timing_constraint=None  locs_specified=off  LOCs={}  io_standard={}  inherit_from_input=off  hdl_port=on  XmcBlockStatus=1  maskContainerNames=group4  block_type=gatewayin  block_config=sysgen:gateway_in_config  block_width_w=590  block_height_w=620  block_width=640  block_height=850
  out_mat_dac1_selx1 : hdlBasic/Gateway In  gui_display_data_type=Fixed-point  arith_type=Unsigned  n_bits=2  bin_pt=0  preci_type=Single  exp_width=8  frac_width=24  rows=1  columns=1  quantization=Truncate  overflow=Wrap  period=hw.t_axi  UseAsADC=off  ADCChannel='1'  interface=AXI4-Lite  automatic_assignment=off  address_offset=ip.offsets.output_mat_cfg + hex2dec('1c')  intf_name=''  intf_description=''  default_value=0  timing_constraint=None  locs_specified=off  LOCs={}  io_standard={}  inherit_from_input=off  hdl_port=on  XmcBlockStatus=1  maskContainerNames=group4  block_type=gatewayin  block_config=sysgen:gateway_in_config  block_width_w=590  block_height_w=620  block_width=640  block_height=850
  out_mat_dac1_selx2 : hdlBasic/Gateway In  gui_display_data_type=Fixed-point  arith_type=Unsigned  n_bits=2  bin_pt=0  preci_type=Single  exp_width=8  frac_width=24  rows=1  columns=1  quantization=Truncate  overflow=Wrap  period=hw.t_axi  UseAsADC=off  ADCChannel='1'  interface=AXI4-Lite  automatic_assignment=off  address_offset=ip.offsets.output_mat_cfg + hex2dec('20')  intf_name=''  intf_description=''  default_value=0  timing_constraint=None  locs_specified=off  LOCs={}  io_standard={}  inherit_from_input=off  hdl_port=on  XmcBlockStatus=1  maskContainerNames=group4  block_type=gatewayin  block_config=sysgen:gateway_in_config  block_width_w=590  block_height_w=620  block_width=640  block_height=850
  out_mat_fac_dac0_xx0 : hdlBasic/Gateway In  gui_display_data_type=Fixed-point  arith_type=Signed (2's comp)  n_bits=dt.const.sz  bin_pt=dt.const.bin  preci_type=Single  exp_width=8  frac_width=24  rows=1  columns=1  quantization=Truncate  overflow=Wrap  period=hw.t_axi  UseAsADC=off  ADCChannel='1'  interface=AXI4-Lite  automatic_assignment=off  address_offset=ip.offsets.output_mat_cfg + hex2dec('0c')  intf_name=''  intf_description=''  default_value=0  timing_constraint=None  locs_specified=off  LOCs={}  io_standard={}  inherit_from_input=off  hdl_port=on  XmcBlockStatus=1  maskContainerNames=group4  block_type=gatewayin  block_config=sysgen:gateway_in_config  block_width_w=590  block_height_w=620  block_width=640  block_height=850
  out_mat_fac_dac0_xx1 : hdlBasic/Gateway In  gui_display_data_type=Fixed-point  arith_type=Signed (2's comp)  n_bits=dt.const.sz  bin_pt=dt.const.bin  preci_type=Single  exp_width=8  frac_width=24  rows=1  columns=1  quantization=Truncate  overflow=Wrap  period=hw.t_axi  UseAsADC=off  ADCChannel='1'  interface=AXI4-Lite  automatic_assignment=off  address_offset=ip.offsets.output_mat_cfg + hex2dec('10')  intf_name=''  intf_description=''  default_value=0  timing_constraint=None  locs_specified=off  LOCs={}  io_standard={}  inherit_from_input=off  hdl_port=on  XmcBlockStatus=1  maskContainerNames=group4  block_type=gatewayin  block_config=sysgen:gateway_in_config  block_width_w=590  block_height_w=620  block_width=640  block_height=850
  out_mat_fac_dac0_xx2 : hdlBasic/Gateway In  gui_display_data_type=Fixed-point  arith_type=Signed (2's comp)  n_bits=dt.const.sz  bin_pt=dt.const.bin  preci_type=Single  exp_width=8  frac_width=24  rows=1  columns=1  quantization=Truncate  overflow=Wrap  period=hw.t_axi  UseAsADC=off  ADCChannel='1'  interface=AXI4-Lite  automatic_assignment=off  address_offset=ip.offsets.output_mat_cfg + hex2dec('14')  intf_name=''  intf_description=''  default_value=0  timing_constraint=None  locs_specified=off  LOCs={}  io_standard={}  inherit_from_input=off  hdl_port=on  XmcBlockStatus=1  maskContainerNames=group4  block_type=gatewayin  block_config=sysgen:gateway_in_config  block_width_w=590  block_height_w=620  block_width=640  block_height=850
  out_mat_fac_dac1_xx0 : hdlBasic/Gateway In  gui_display_data_type=Fixed-point  arith_type=Signed (2's comp)  n_bits=dt.const.sz  bin_pt=dt.const.bin  preci_type=Single  exp_width=8  frac_width=24  rows=1  columns=1  quantization=Truncate  overflow=Wrap  period=hw.t_axi  UseAsADC=off  ADCChannel='1'  interface=AXI4-Lite  automatic_assignment=off  address_offset=ip.offsets.output_mat_cfg + hex2dec('24')  intf_name=''  intf_description=''  default_value=0  timing_constraint=None  locs_specified=off  LOCs={}  io_standard={}  inherit_from_input=off  hdl_port=on  XmcBlockStatus=1  maskContainerNames=group4  block_type=gatewayin  block_config=sysgen:gateway_in_config  block_width_w=590  block_height_w=620  block_width=640  block_height=850
  out_mat_fac_dac1_xx1 : hdlBasic/Gateway In  gui_display_data_type=Fixed-point  arith_type=Signed (2's comp)  n_bits=dt.const.sz  bin_pt=dt.const.bin  preci_type=Single  exp_width=8  frac_width=24  rows=1  columns=1  quantization=Truncate  overflow=Wrap  period=hw.t_axi  UseAsADC=off  ADCChannel='1'  interface=AXI4-Lite  automatic_assignment=off  address_offset=ip.offsets.output_mat_cfg + hex2dec('28')  intf_name=''  intf_description=''  default_value=0  timing_constraint=None  locs_specified=off  LOCs={}  io_standard={}  inherit_from_input=off  hdl_port=on  XmcBlockStatus=1  maskContainerNames=group4  block_type=gatewayin  block_config=sysgen:gateway_in_config  block_width_w=590  block_height_w=620  block_width=640  block_height=850
  out_mat_fac_dac1_xx2 : hdlBasic/Gateway In  gui_display_data_type=Fixed-point  arith_type=Signed (2's comp)  n_bits=dt.const.sz  bin_pt=dt.const.bin  preci_type=Single  exp_width=8  frac_width=24  rows=1  columns=1  quantization=Truncate  overflow=Wrap  period=hw.t_axi  UseAsADC=off  ADCChannel='1'  interface=AXI4-Lite  automatic_assignment=off  address_offset=ip.offsets.output_mat_cfg + hex2dec('2c')  intf_name=''  intf_description=''  default_value=0  timing_constraint=None  locs_specified=off  LOCs={}  io_standard={}  inherit_from_input=off  hdl_port=on  XmcBlockStatus=1  maskContainerNames=group4  block_type=gatewayin  block_config=sysgen:gateway_in_config  block_width_w=590  block_height_w=620  block_width=640  block_height=850
  out_mat_nlf_dac0_xx0_en : hdlBasic/Gateway In  gui_display_data_type=Boolean  arith_type=Boolean  n_bits=8  bin_pt=0  preci_type=Single  exp_width=8  frac_width=24  rows=1  columns=1  quantization=Truncate  overflow=Wrap  period=hw.t_axi  UseAsADC=off  ADCChannel='1'  interface=AXI4-Lite  automatic_assignment=off  address_offset=ip.offsets.output_mat_cfg + hex2dec('30')  intf_name=''  intf_description=''  default_value=0  timing_constraint=None  locs_specified=off  LOCs={}  io_standard={}  inherit_from_input=off  hdl_port=on  XmcBlockStatus=1  maskContainerNames=group4  block_type=gatewayin  block_config=sysgen:gateway_in_config  block_width_w=590  block_height_w=620  block_width=640  block_height=850
  out_mat_nlf_dac0_xx0_gain : hdlBasic/Gateway In  gui_display_data_type=Fixed-point  arith_type=Signed (2's comp)  n_bits=dt.const.sz  bin_pt=dt.const.bin  preci_type=Single  exp_width=8  frac_width=24  rows=1  columns=1  quantization=Truncate  overflow=Wrap  period=hw.t_axi  UseAsADC=off  ADCChannel='1'  interface=AXI4-Lite  automatic_assignment=off  address_offset=ip.offsets.output_mat_cfg + hex2dec('38')  intf_name=''  intf_description=''  default_value=0  timing_constraint=None  locs_specified=off  LOCs={}  io_standard={}  inherit_from_input=off  hdl_port=on  XmcBlockStatus=1  maskContainerNames=group4  block_type=gatewayin  block_config=sysgen:gateway_in_config  block_width_w=590  block_height_w=620  block_width=640  block_height=850
  out_mat_nlf_dac0_xx0_presc : hdlBasic/Gateway In  gui_display_data_type=Fixed-point  arith_type=Signed (2's comp)  n_bits=dt.const.sz  bin_pt=dt.const.bin  preci_type=Single  exp_width=8  frac_width=24  rows=1  columns=1  quantization=Truncate  overflow=Wrap  period=hw.t_axi  UseAsADC=off  ADCChannel='1'  interface=AXI4-Lite  automatic_assignment=off  address_offset=ip.offsets.output_mat_cfg + hex2dec('34')  intf_name=''  intf_description=''  default_value=0  timing_constraint=None  locs_specified=off  LOCs={}  io_standard={}  inherit_from_input=off  hdl_port=on  XmcBlockStatus=1  maskContainerNames=group4  block_type=gatewayin  block_config=sysgen:gateway_in_config  block_width_w=590  block_height_w=620  block_width=640  block_height=850
  out_mat_nlf_dac0_xx1_en : hdlBasic/Gateway In  gui_display_data_type=Boolean  arith_type=Boolean  n_bits=8  bin_pt=0  preci_type=Single  exp_width=8  frac_width=24  rows=1  columns=1  quantization=Truncate  overflow=Wrap  period=hw.t_axi  UseAsADC=off  ADCChannel='1'  interface=AXI4-Lite  automatic_assignment=off  address_offset=ip.offsets.output_mat_cfg + hex2dec('3c')  intf_name=''  intf_description=''  default_value=0  timing_constraint=None  locs_specified=off  LOCs={}  io_standard={}  inherit_from_input=off  hdl_port=on  XmcBlockStatus=1  maskContainerNames=group4  block_type=gatewayin  block_config=sysgen:gateway_in_config  block_width_w=590  block_height_w=620  block_width=640  block_height=850
  out_mat_nlf_dac0_xx1_gain : hdlBasic/Gateway In  gui_display_data_type=Fixed-point  arith_type=Signed (2's comp)  n_bits=dt.const.sz  bin_pt=dt.const.bin  preci_type=Single  exp_width=8  frac_width=24  rows=1  columns=1  quantization=Truncate  overflow=Wrap  period=hw.t_axi  UseAsADC=off  ADCChannel='1'  interface=AXI4-Lite  automatic_assignment=off  address_offset=ip.offsets.output_mat_cfg + hex2dec('44')  intf_name=''  intf_description=''  default_value=0  timing_constraint=None  locs_specified=off  LOCs={}  io_standard={}  inherit_from_input=off  hdl_port=on  XmcBlockStatus=1  maskContainerNames=group4  block_type=gatewayin  block_config=sysgen:gateway_in_config  block_width_w=590  block_height_w=620  block_width=640  block_height=850
  out_mat_nlf_dac0_xx1_presc : hdlBasic/Gateway In  gui_display_data_type=Fixed-point  arith_type=Signed (2's comp)  n_bits=dt.const.sz  bin_pt=dt.const.bin  preci_type=Single  exp_width=8  frac_width=24  rows=1  columns=1  quantization=Truncate  overflow=Wrap  period=hw.t_axi  UseAsADC=off  ADCChannel='1'  interface=AXI4-Lite  automatic_assignment=off  address_offset=ip.offsets.output_mat_cfg + hex2dec('40')  intf_name=''  intf_description=''  default_value=0  timing_constraint=None  locs_specified=off  LOCs={}  io_standard={}  inherit_from_input=off  hdl_port=on  XmcBlockStatus=1  maskContainerNames=group4  block_type=gatewayin  block_config=sysgen:gateway_in_config  block_width_w=590  block_height_w=620  block_width=640  block_height=850
  out_mat_nlf_dac0_xx2_en : hdlBasic/Gateway In  gui_display_data_type=Boolean  arith_type=Boolean  n_bits=8  bin_pt=0  preci_type=Single  exp_width=8  frac_width=24  rows=1  columns=1  quantization=Truncate  overflow=Wrap  period=hw.t_axi  UseAsADC=off  ADCChannel='1'  interface=AXI4-Lite  automatic_assignment=off  address_offset=ip.offsets.output_mat_cfg + hex2dec('48')  intf_name=''  intf_description=''  default_value=0  timing_constraint=None  locs_specified=off  LOCs={}  io_standard={}  inherit_from_input=off  hdl_port=on  XmcBlockStatus=1  maskContainerNames=group4  block_type=gatewayin  block_config=sysgen:gateway_in_config  block_width_w=590  block_height_w=620  block_width=640  block_height=850
  out_mat_nlf_dac0_xx2_gain : hdlBasic/Gateway In  gui_display_data_type=Fixed-point  arith_type=Signed (2's comp)  n_bits=dt.const.sz  bin_pt=dt.const.bin  preci_type=Single  exp_width=8  frac_width=24  rows=1  columns=1  quantization=Truncate  overflow=Wrap  period=hw.t_axi  UseAsADC=off  ADCChannel='1'  interface=AXI4-Lite  automatic_assignment=off  address_offset=ip.offsets.output_mat_cfg + hex2dec('50')  intf_name=''  intf_description=''  default_value=0  timing_constraint=None  locs_specified=off  LOCs={}  io_standard={}  inherit_from_input=off  hdl_port=on  XmcBlockStatus=1  maskContainerNames=group4  block_type=gatewayin  block_config=sysgen:gateway_in_config  block_width_w=590  block_height_w=620  block_width=640  block_height=850
  out_mat_nlf_dac0_xx2_presc : hdlBasic/Gateway In  gui_display_data_type=Fixed-point  arith_type=Signed (2's comp)  n_bits=dt.const.sz  bin_pt=dt.const.bin  preci_type=Single  exp_width=8  frac_width=24  rows=1  columns=1  quantization=Truncate  overflow=Wrap  period=hw.t_axi  UseAsADC=off  ADCChannel='1'  interface=AXI4-Lite  automatic_assignment=off  address_offset=ip.offsets.output_mat_cfg + hex2dec('4c')  intf_name=''  intf_description=''  default_value=0  timing_constraint=None  locs_specified=off  LOCs={}  io_standard={}  inherit_from_input=off  hdl_port=on  XmcBlockStatus=1  maskContainerNames=group4  block_type=gatewayin  block_config=sysgen:gateway_in_config  block_width_w=590  block_height_w=620  block_width=640  block_height=850
  out_mat_nlf_dac1_xx0_en : hdlBasic/Gateway In  gui_display_data_type=Boolean  arith_type=Boolean  n_bits=8  bin_pt=0  preci_type=Single  exp_width=8  frac_width=24  rows=1  columns=1  quantization=Truncate  overflow=Wrap  period=hw.t_axi  UseAsADC=off  ADCChannel='1'  interface=AXI4-Lite  automatic_assignment=off  address_offset=ip.offsets.output_mat_cfg + hex2dec('54')  intf_name=''  intf_description=''  default_value=0  timing_constraint=None  locs_specified=off  LOCs={}  io_standard={}  inherit_from_input=off  hdl_port=on  XmcBlockStatus=1  maskContainerNames=group4  block_type=gatewayin  block_config=sysgen:gateway_in_config  block_width_w=590  block_height_w=620  block_width=640  block_height=850
  out_mat_nlf_dac1_xx0_gain : hdlBasic/Gateway In  gui_display_data_type=Fixed-point  arith_type=Signed (2's comp)  n_bits=dt.const.sz  bin_pt=dt.const.bin  preci_type=Single  exp_width=8  frac_width=24  rows=1  columns=1  quantization=Truncate  overflow=Wrap  period=hw.t_axi  UseAsADC=off  ADCChannel='1'  interface=AXI4-Lite  automatic_assignment=off  address_offset=ip.offsets.output_mat_cfg + hex2dec('5c')  intf_name=''  intf_description=''  default_value=0  timing_constraint=None  locs_specified=off  LOCs={}  io_standard={}  inherit_from_input=off  hdl_port=on  XmcBlockStatus=1  maskContainerNames=group4  block_type=gatewayin  block_config=sysgen:gateway_in_config  block_width_w=590  block_height_w=620  block_width=640  block_height=850
  out_mat_nlf_dac1_xx0_presc : hdlBasic/Gateway In  gui_display_data_type=Fixed-point  arith_type=Signed (2's comp)  n_bits=dt.const.sz  bin_pt=dt.const.bin  preci_type=Single  exp_width=8  frac_width=24  rows=1  columns=1  quantization=Truncate  overflow=Wrap  period=hw.t_axi  UseAsADC=off  ADCChannel='1'  interface=AXI4-Lite  automatic_assignment=off  address_offset=ip.offsets.output_mat_cfg + hex2dec('58')  intf_name=''  intf_description=''  default_value=0  timing_constraint=None  locs_specified=off  LOCs={}  io_standard={}  inherit_from_input=off  hdl_port=on  XmcBlockStatus=1  maskContainerNames=group4  block_type=gatewayin  block_config=sysgen:gateway_in_config  block_width_w=590  block_height_w=620  block_width=640  block_height=850
  out_mat_nlf_dac1_xx1_en : hdlBasic/Gateway In  gui_display_data_type=Boolean  arith_type=Boolean  n_bits=8  bin_pt=0  preci_type=Single  exp_width=8  frac_width=24  rows=1  columns=1  quantization=Truncate  overflow=Wrap  period=hw.t_axi  UseAsADC=off  ADCChannel='1'  interface=AXI4-Lite  automatic_assignment=off  address_offset=ip.offsets.output_mat_cfg + hex2dec('60')  intf_name=''  intf_description=''  default_value=0  timing_constraint=None  locs_specified=off  LOCs={}  io_standard={}  inherit_from_input=off  hdl_port=on  XmcBlockStatus=1  maskContainerNames=group4  block_type=gatewayin  block_config=sysgen:gateway_in_config  block_width_w=590  block_height_w=620  block_width=640  block_height=850
  out_mat_nlf_dac1_xx1_gain : hdlBasic/Gateway In  gui_display_data_type=Fixed-point  arith_type=Signed (2's comp)  n_bits=dt.const.sz  bin_pt=dt.const.bin  preci_type=Single  exp_width=8  frac_width=24  rows=1  columns=1  quantization=Truncate  overflow=Wrap  period=hw.t_axi  UseAsADC=off  ADCChannel='1'  interface=AXI4-Lite  automatic_assignment=off  address_offset=ip.offsets.output_mat_cfg + hex2dec('68')  intf_name=''  intf_description=''  default_value=0  timing_constraint=None  locs_specified=off  LOCs={}  io_standard={}  inherit_from_input=off  hdl_port=on  XmcBlockStatus=1  maskContainerNames=group4  block_type=gatewayin  block_config=sysgen:gateway_in_config  block_width_w=590  block_height_w=620  block_width=640  block_height=850
  out_mat_nlf_dac1_xx1_presc : hdlBasic/Gateway In  gui_display_data_type=Fixed-point  arith_type=Signed (2's comp)  n_bits=dt.const.sz  bin_pt=dt.const.bin  preci_type=Single  exp_width=8  frac_width=24  rows=1  columns=1  quantization=Truncate  overflow=Wrap  period=hw.t_axi  UseAsADC=off  ADCChannel='1'  interface=AXI4-Lite  automatic_assignment=off  address_offset=ip.offsets.output_mat_cfg + hex2dec('64')  intf_name=''  intf_description=''  default_value=0  timing_constraint=None  locs_specified=off  LOCs={}  io_standard={}  inherit_from_input=off  hdl_port=on  XmcBlockStatus=1  maskContainerNames=group4  block_type=gatewayin  block_config=sysgen:gateway_in_config  block_width_w=590  block_height_w=620  block_width=640  block_height=850
  out_mat_nlf_dac1_xx2_en : hdlBasic/Gateway In  gui_display_data_type=Boolean  arith_type=Boolean  n_bits=8  bin_pt=0  preci_type=Single  exp_width=8  frac_width=24  rows=1  columns=1  quantization=Truncate  overflow=Wrap  period=hw.t_axi  UseAsADC=off  ADCChannel='1'  interface=AXI4-Lite  automatic_assignment=off  address_offset=ip.offsets.output_mat_cfg + hex2dec('6c')  intf_name=''  intf_description=''  default_value=0  timing_constraint=None  locs_specified=off  LOCs={}  io_standard={}  inherit_from_input=off  hdl_port=on  XmcBlockStatus=1  maskContainerNames=group4  block_type=gatewayin  block_config=sysgen:gateway_in_config  block_width_w=590  block_height_w=620  block_width=640  block_height=850
  out_mat_nlf_dac1_xx2_gain : hdlBasic/Gateway In  gui_display_data_type=Fixed-point  arith_type=Signed (2's comp)  n_bits=dt.const.sz  bin_pt=dt.const.bin  preci_type=Single  exp_width=8  frac_width=24  rows=1  columns=1  quantization=Truncate  overflow=Wrap  period=hw.t_axi  UseAsADC=off  ADCChannel='1'  interface=AXI4-Lite  automatic_assignment=off  address_offset=ip.offsets.output_mat_cfg + hex2dec('74')  intf_name=''  intf_description=''  default_value=0  timing_constraint=None  locs_specified=off  LOCs={}  io_standard={}  inherit_from_input=off  hdl_port=on  XmcBlockStatus=1  maskContainerNames=group4  block_type=gatewayin  block_config=sysgen:gateway_in_config  block_width_w=590  block_height_w=620  block_width=640  block_height=850
  out_mat_nlf_dac1_xx2_presc : hdlBasic/Gateway In  gui_display_data_type=Fixed-point  arith_type=Signed (2's comp)  n_bits=dt.const.sz  bin_pt=dt.const.bin  preci_type=Single  exp_width=8  frac_width=24  rows=1  columns=1  quantization=Truncate  overflow=Wrap  period=hw.t_axi  UseAsADC=off  ADCChannel='1'  interface=AXI4-Lite  automatic_assignment=off  address_offset=ip.offsets.output_mat_cfg + hex2dec('70')  intf_name=''  intf_description=''  default_value=0  timing_constraint=None  locs_specified=off  LOCs={}  io_standard={}  inherit_from_input=off  hdl_port=on  XmcBlockStatus=1  maskContainerNames=group4  block_type=gatewayin  block_config=sysgen:gateway_in_config  block_width_w=590  block_height_w=620  block_width=640  block_height=850
  slice0_u_gain : hdlBasic/Gateway In  gui_display_data_type=Fixed-point  arith_type=Signed (2's comp)  n_bits=dt.const.sz  bin_pt=dt.const.bin  preci_type=Single  exp_width=8  frac_width=24  rows=1  columns=1  quantization=Truncate  overflow=Wrap  period=hw.t_axi  UseAsADC=off  ADCChannel='1'  interface=AXI4-Lite  automatic_assignment=off  address_offset=ip.offsets.slice0_cfg + hex2dec('24')  intf_name=''  intf_description=''  default_value=0  timing_constraint=None  locs_specified=off  LOCs={}  io_standard={}  inherit_from_input=off  hdl_port=on  XmcBlockStatus=1  maskContainerNames=group4  block_type=gatewayin  block_config=sysgen:gateway_in_config  block_width_w=590  block_height_w=620  block_width=640  block_height=850
  slice0_u_mux : hdlBasic/Gateway In  gui_display_data_type=Boolean  arith_type=Boolean  n_bits=8  bin_pt=0  preci_type=Single  exp_width=8  frac_width=24  rows=1  columns=1  quantization=Truncate  overflow=Wrap  period=hw.t_axi  UseAsADC=off  ADCChannel='1'  interface=AXI4-Lite  automatic_assignment=off  address_offset=ip.offsets.slice0_cfg + hex2dec('20')  intf_name=''  intf_description=''  default_value=0  timing_constraint=None  locs_specified=off  LOCs={}  io_standard={}  inherit_from_input=off  hdl_port=on  XmcBlockStatus=1  maskContainerNames=group4  block_type=gatewayin  block_config=sysgen:gateway_in_config  block_width_w=590  block_height_w=620  block_width=640  block_height=850
  slice0_u_nlf_gain : hdlBasic/Gateway In  gui_display_data_type=Fixed-point  arith_type=Signed (2's comp)  n_bits=dt.const.sz  bin_pt=dt.const.bin  preci_type=Single  exp_width=8  frac_width=24  rows=1  columns=1  quantization=Truncate  overflow=Wrap  period=hw.t_axi  UseAsADC=off  ADCChannel='1'  interface=AXI4-Lite  automatic_assignment=off  address_offset=ip.offsets.slice0_cfg + hex2dec('2c')  intf_name=''  intf_description=''  default_value=0  timing_constraint=None  locs_specified=off  LOCs={}  io_standard={}  inherit_from_input=off  hdl_port=on  XmcBlockStatus=1  maskContainerNames=group4  block_type=gatewayin  block_config=sysgen:gateway_in_config  block_width_w=590  block_height_w=620  block_width=640  block_height=850
  slice0_u_nlf_presc : hdlBasic/Gateway In  gui_display_data_type=Fixed-point  arith_type=Signed (2's comp)  n_bits=dt.const.sz  bin_pt=dt.const.bin  preci_type=Single  exp_width=8  frac_width=24  rows=1  columns=1  quantization=Truncate  overflow=Wrap  period=hw.t_axi  UseAsADC=off  ADCChannel='1'  interface=AXI4-Lite  automatic_assignment=off  address_offset=ip.offsets.slice0_cfg + hex2dec('28')  intf_name=''  intf_description=''  default_value=0  timing_constraint=None  locs_specified=off  LOCs={}  io_standard={}  inherit_from_input=off  hdl_port=on  XmcBlockStatus=1  maskContainerNames=group4  block_type=gatewayin  block_config=sysgen:gateway_in_config  block_width_w=590  block_height_w=620  block_width=640  block_height=850
  slice0_x_gain : hdlBasic/Gateway In  gui_display_data_type=Fixed-point  arith_type=Signed (2's comp)  n_bits=dt.const.sz  bin_pt=dt.const.bin  preci_type=Single  exp_width=8  frac_width=24  rows=1  columns=1  quantization=Truncate  overflow=Wrap  period=hw.t_axi  UseAsADC=off  ADCChannel='1'  interface=AXI4-Lite  automatic_assignment=off  address_offset=ip.offsets.slice0_cfg + hex2dec('04')  intf_name=''  intf_description=''  default_value=0  timing_constraint=None  locs_specified=off  LOCs={}  io_standard={}  inherit_from_input=off  hdl_port=on  XmcBlockStatus=1  maskContainerNames=group4  block_type=gatewayin  block_config=sysgen:gateway_in_config  block_width_w=590  block_height_w=620  block_width=640  block_height=850
  slice0_x_mux : hdlBasic/Gateway In  gui_display_data_type=Boolean  arith_type=Boolean  n_bits=8  bin_pt=0  preci_type=Single  exp_width=8  frac_width=24  rows=1  columns=1  quantization=Truncate  overflow=Wrap  period=hw.t_axi  UseAsADC=off  ADCChannel='1'  interface=AXI4-Lite  automatic_assignment=off  address_offset=ip.offsets.slice0_cfg + hex2dec('00')  intf_name=''  intf_description=''  default_value=0  timing_constraint=None  locs_specified=off  LOCs={}  io_standard={}  inherit_from_input=off  hdl_port=on  XmcBlockStatus=1  maskContainerNames=group4  block_type=gatewayin  block_config=sysgen:gateway_in_config  block_width_w=590  block_height_w=620  block_width=640  block_height=850
  slice0_x_nlf_gain : hdlBasic/Gateway In  gui_display_data_type=Fixed-point  arith_type=Signed (2's comp)  n_bits=dt.const.sz  bin_pt=dt.const.bin  preci_type=Single  exp_width=8  frac_width=24  rows=1  columns=1  quantization=Truncate  overflow=Wrap  period=hw.t_axi  UseAsADC=off  ADCChannel='1'  interface=AXI4-Lite  automatic_assignment=off  address_offset=ip.offsets.slice0_cfg + hex2dec('0c')  intf_name=''  intf_description=''  default_value=0  timing_constraint=None  locs_specified=off  LOCs={}  io_standard={}  inherit_from_input=off  hdl_port=on  XmcBlockStatus=1  maskContainerNames=group4  block_type=gatewayin  block_config=sysgen:gateway_in_config  block_width_w=590  block_height_w=620  block_width=640  block_height=850
  slice0_x_nlf_presc : hdlBasic/Gateway In  gui_display_data_type=Fixed-point  arith_type=Signed (2's comp)  n_bits=dt.const.sz  bin_pt=dt.const.bin  preci_type=Single  exp_width=8  frac_width=24  rows=1  columns=1  quantization=Truncate  overflow=Wrap  period=hw.t_axi  UseAsADC=off  ADCChannel='1'  interface=AXI4-Lite  automatic_assignment=off  address_offset=ip.offsets.slice0_cfg + hex2dec('08')  intf_name=''  intf_description=''  default_value=0  timing_constraint=None  locs_specified=off  LOCs={}  io_standard={}  inherit_from_input=off  hdl_port=on  XmcBlockStatus=1  maskContainerNames=group4  block_type=gatewayin  block_config=sysgen:gateway_in_config  block_width_w=590  block_height_w=620  block_width=640  block_height=850
  slice0_x_presc_mul : hdlBasic/Gateway In  gui_display_data_type=Fixed-point  arith_type=Signed (2's comp)  n_bits=dt.const.sz  bin_pt=dt.const.bin  preci_type=Single  exp_width=8  frac_width=24  rows=1  columns=1  quantization=Truncate  overflow=Wrap  period=hw.t_axi  UseAsADC=off  ADCChannel='1'  interface=AXI4-Lite  automatic_assignment=off  address_offset=ip.offsets.slice0_cfg + hex2dec('3c')  intf_name=''  intf_description=''  default_value=0  timing_constraint=None  locs_specified=off  LOCs={}  io_standard={}  inherit_from_input=off  hdl_port=on  XmcBlockStatus=1  maskContainerNames=group4  block_type=gatewayin  block_config=sysgen:gateway_in_config  block_width_w=590  block_height_w=620  block_width=640  block_height=850
  slice0_x_presc_shift : hdlBasic/Gateway In  gui_display_data_type=Fixed-point  arith_type=Unsigned  n_bits=5  bin_pt=0  preci_type=Single  exp_width=8  frac_width=24  rows=1  columns=1  quantization=Truncate  overflow=Wrap  period=hw.t_axi  UseAsADC=off  ADCChannel='1'  interface=AXI4-Lite  automatic_assignment=off  address_offset=ip.offsets.slice0_cfg + hex2dec('38')  intf_name=''  intf_description=''  default_value=0  timing_constraint=None  locs_specified=off  LOCs={}  io_standard={}  inherit_from_input=off  hdl_port=on  XmcBlockStatus=1  maskContainerNames=group4  block_type=gatewayin  block_config=sysgen:gateway_in_config  block_width_w=590  block_height_w=620  block_width=640  block_height=850
  slice0_xd_gain : hdlBasic/Gateway In  gui_display_data_type=Fixed-point  arith_type=Signed (2's comp)  n_bits=dt.const.sz  bin_pt=dt.const.bin  preci_type=Single  exp_width=8  frac_width=24  rows=1  columns=1  quantization=Truncate  overflow=Wrap  period=hw.t_axi  UseAsADC=off  ADCChannel='1'  interface=AXI4-Lite  automatic_assignment=off  address_offset=ip.offsets.slice0_cfg + hex2dec('14')  intf_name=''  intf_description=''  default_value=0  timing_constraint=None  locs_specified=off  LOCs={}  io_standard={}  inherit_from_input=off  hdl_port=on  XmcBlockStatus=1  maskContainerNames=group4  block_type=gatewayin  block_config=sysgen:gateway_in_config  block_width_w=590  block_height_w=620  block_width=640  block_height=850
  slice0_xd_mux : hdlBasic/Gateway In  gui_display_data_type=Boolean  arith_type=Boolean  n_bits=8  bin_pt=0  preci_type=Single  exp_width=8  frac_width=24  rows=1  columns=1  quantization=Truncate  overflow=Wrap  period=hw.t_axi  UseAsADC=off  ADCChannel='1'  interface=AXI4-Lite  automatic_assignment=off  address_offset=ip.offsets.slice0_cfg + hex2dec('10')  intf_name=''  intf_description=''  default_value=0  timing_constraint=None  locs_specified=off  LOCs={}  io_standard={}  inherit_from_input=off  hdl_port=on  XmcBlockStatus=1  maskContainerNames=group4  block_type=gatewayin  block_config=sysgen:gateway_in_config  block_width_w=590  block_height_w=620  block_width=640  block_height=850
  slice0_xd_nlf_gain : hdlBasic/Gateway In  gui_display_data_type=Fixed-point  arith_type=Signed (2's comp)  n_bits=dt.const.sz  bin_pt=dt.const.bin  preci_type=Single  exp_width=8  frac_width=24  rows=1  columns=1  quantization=Truncate  overflow=Wrap  period=hw.t_axi  UseAsADC=off  ADCChannel='1'  interface=AXI4-Lite  automatic_assignment=off  address_offset=ip.offsets.slice0_cfg + hex2dec('1c')  intf_name=''  intf_description=''  default_value=0  timing_constraint=None  locs_specified=off  LOCs={}  io_standard={}  inherit_from_input=off  hdl_port=on  XmcBlockStatus=1  maskContainerNames=group4  block_type=gatewayin  block_config=sysgen:gateway_in_config  block_width_w=590  block_height_w=620  block_width=640  block_height=850
  slice0_xd_nlf_presc : hdlBasic/Gateway In  gui_display_data_type=Fixed-point  arith_type=Signed (2's comp)  n_bits=dt.const.sz  bin_pt=dt.const.bin  preci_type=Single  exp_width=8  frac_width=24  rows=1  columns=1  quantization=Truncate  overflow=Wrap  period=hw.t_axi  UseAsADC=off  ADCChannel='1'  interface=AXI4-Lite  automatic_assignment=off  address_offset=ip.offsets.slice0_cfg + hex2dec('18')  intf_name=''  intf_description=''  default_value=0  timing_constraint=None  locs_specified=off  LOCs={}  io_standard={}  inherit_from_input=off  hdl_port=on  XmcBlockStatus=1  maskContainerNames=group4  block_type=gatewayin  block_config=sysgen:gateway_in_config  block_width_w=590  block_height_w=620  block_width=640  block_height=850
  slice0_xd_presc_mul : hdlBasic/Gateway In  gui_display_data_type=Fixed-point  arith_type=Signed (2's comp)  n_bits=dt.const.sz  bin_pt=dt.const.bin  preci_type=Single  exp_width=8  frac_width=24  rows=1  columns=1  quantization=Truncate  overflow=Wrap  period=hw.t_axi  UseAsADC=off  ADCChannel='1'  interface=AXI4-Lite  automatic_assignment=off  address_offset=ip.offsets.slice0_cfg + hex2dec('34')  intf_name=''  intf_description=''  default_value=0  timing_constraint=None  locs_specified=off  LOCs={}  io_standard={}  inherit_from_input=off  hdl_port=on  XmcBlockStatus=1  maskContainerNames=group4  block_type=gatewayin  block_config=sysgen:gateway_in_config  block_width_w=590  block_height_w=620  block_width=640  block_height=850
  slice0_xd_presc_shift : hdlBasic/Gateway In  gui_display_data_type=Fixed-point  arith_type=Unsigned  n_bits=5  bin_pt=0  preci_type=Single  exp_width=8  frac_width=24  rows=1  columns=1  quantization=Truncate  overflow=Wrap  period=hw.t_axi  UseAsADC=off  ADCChannel='1'  interface=AXI4-Lite  automatic_assignment=off  address_offset=ip.offsets.slice0_cfg + hex2dec('30')  intf_name=''  intf_description=''  default_value=0  timing_constraint=None  locs_specified=off  LOCs={}  io_standard={}  inherit_from_input=off  hdl_port=on  XmcBlockStatus=1  maskContainerNames=group4  block_type=gatewayin  block_config=sysgen:gateway_in_config  block_width_w=590  block_height_w=620  block_width=640  block_height=850
  slice1_u_gain : hdlBasic/Gateway In  gui_display_data_type=Fixed-point  arith_type=Signed (2's comp)  n_bits=dt.const.sz  bin_pt=dt.const.bin  preci_type=Single  exp_width=8  frac_width=24  rows=1  columns=1  quantization=Truncate  overflow=Wrap  period=hw.t_axi  UseAsADC=off  ADCChannel='1'  interface=AXI4-Lite  automatic_assignment=off  address_offset=ip.offsets.slice1_cfg + hex2dec('24')  intf_name=''  intf_description=''  default_value=0  timing_constraint=None  locs_specified=off  LOCs={}  io_standard={}  inherit_from_input=off  hdl_port=on  XmcBlockStatus=1  maskContainerNames=group4  block_type=gatewayin  block_config=sysgen:gateway_in_config  block_width_w=590  block_height_w=620  block_width=640  block_height=850
  slice1_u_mux : hdlBasic/Gateway In  gui_display_data_type=Boolean  arith_type=Boolean  n_bits=8  bin_pt=0  preci_type=Single  exp_width=8  frac_width=24  rows=1  columns=1  quantization=Truncate  overflow=Wrap  period=hw.t_axi  UseAsADC=off  ADCChannel='1'  interface=AXI4-Lite  automatic_assignment=off  address_offset=ip.offsets.slice1_cfg + hex2dec('20')  intf_name=''  intf_description=''  default_value=0  timing_constraint=None  locs_specified=off  LOCs={}  io_standard={}  inherit_from_input=off  hdl_port=on  XmcBlockStatus=1  maskContainerNames=group4  block_type=gatewayin  block_config=sysgen:gateway_in_config  block_width_w=590  block_height_w=620  block_width=640  block_height=850
  slice1_u_nlf_gain : hdlBasic/Gateway In  gui_display_data_type=Fixed-point  arith_type=Signed (2's comp)  n_bits=dt.const.sz  bin_pt=dt.const.bin  preci_type=Single  exp_width=8  frac_width=24  rows=1  columns=1  quantization=Truncate  overflow=Wrap  period=hw.t_axi  UseAsADC=off  ADCChannel='1'  interface=AXI4-Lite  automatic_assignment=off  address_offset=ip.offsets.slice1_cfg + hex2dec('2c')  intf_name=''  intf_description=''  default_value=0  timing_constraint=None  locs_specified=off  LOCs={}  io_standard={}  inherit_from_input=off  hdl_port=on  XmcBlockStatus=1  maskContainerNames=group4  block_type=gatewayin  block_config=sysgen:gateway_in_config  block_width_w=590  block_height_w=620  block_width=640  block_height=850
  slice1_u_nlf_presc : hdlBasic/Gateway In  gui_display_data_type=Fixed-point  arith_type=Signed (2's comp)  n_bits=dt.const.sz  bin_pt=dt.const.bin  preci_type=Single  exp_width=8  frac_width=24  rows=1  columns=1  quantization=Truncate  overflow=Wrap  period=hw.t_axi  UseAsADC=off  ADCChannel='1'  interface=AXI4-Lite  automatic_assignment=off  address_offset=ip.offsets.slice1_cfg + hex2dec('28')  intf_name=''  intf_description=''  default_value=0  timing_constraint=None  locs_specified=off  LOCs={}  io_standard={}  inherit_from_input=off  hdl_port=on  XmcBlockStatus=1  maskContainerNames=group4  block_type=gatewayin  block_config=sysgen:gateway_in_config  block_width_w=590  block_height_w=620  block_width=640  block_height=850
  slice1_x_gain : hdlBasic/Gateway In  gui_display_data_type=Fixed-point  arith_type=Signed (2's comp)  n_bits=dt.const.sz  bin_pt=dt.const.bin  preci_type=Single  exp_width=8  frac_width=24  rows=1  columns=1  quantization=Truncate  overflow=Wrap  period=hw.t_axi  UseAsADC=off  ADCChannel='1'  interface=AXI4-Lite  automatic_assignment=off  address_offset=ip.offsets.slice1_cfg + hex2dec('04')  intf_name=''  intf_description=''  default_value=0  timing_constraint=None  locs_specified=off  LOCs={}  io_standard={}  inherit_from_input=off  hdl_port=on  XmcBlockStatus=1  maskContainerNames=group4  block_type=gatewayin  block_config=sysgen:gateway_in_config  block_width_w=590  block_height_w=620  block_width=640  block_height=850
  slice1_x_mux : hdlBasic/Gateway In  gui_display_data_type=Boolean  arith_type=Boolean  n_bits=8  bin_pt=0  preci_type=Single  exp_width=8  frac_width=24  rows=1  columns=1  quantization=Truncate  overflow=Wrap  period=hw.t_axi  UseAsADC=off  ADCChannel='1'  interface=AXI4-Lite  automatic_assignment=off  address_offset=ip.offsets.slice1_cfg + hex2dec('00')  intf_name=''  intf_description=''  default_value=0  timing_constraint=None  locs_specified=off  LOCs={}  io_standard={}  inherit_from_input=off  hdl_port=on  XmcBlockStatus=1  maskContainerNames=group4  block_type=gatewayin  block_config=sysgen:gateway_in_config  block_width_w=590  block_height_w=620  block_width=640  block_height=850
  slice1_x_nlf_gain : hdlBasic/Gateway In  gui_display_data_type=Fixed-point  arith_type=Signed (2's comp)  n_bits=dt.const.sz  bin_pt=dt.const.bin  preci_type=Single  exp_width=8  frac_width=24  rows=1  columns=1  quantization=Truncate  overflow=Wrap  period=hw.t_axi  UseAsADC=off  ADCChannel='1'  interface=AXI4-Lite  automatic_assignment=off  address_offset=ip.offsets.slice1_cfg + hex2dec('0c')  intf_name=''  intf_description=''  default_value=0  timing_constraint=None  locs_specified=off  LOCs={}  io_standard={}  inherit_from_input=off  hdl_port=on  XmcBlockStatus=1  maskContainerNames=group4  block_type=gatewayin  block_config=sysgen:gateway_in_config  block_width_w=590  block_height_w=620  block_width=640  block_height=850
  slice1_x_nlf_presc : hdlBasic/Gateway In  gui_display_data_type=Fixed-point  arith_type=Signed (2's comp)  n_bits=dt.const.sz  bin_pt=dt.const.bin  preci_type=Single  exp_width=8  frac_width=24  rows=1  columns=1  quantization=Truncate  overflow=Wrap  period=hw.t_axi  UseAsADC=off  ADCChannel='1'  interface=AXI4-Lite  automatic_assignment=off  address_offset=ip.offsets.slice1_cfg + hex2dec('08')  intf_name=''  intf_description=''  default_value=0  timing_constraint=None  locs_specified=off  LOCs={}  io_standard={}  inherit_from_input=off  hdl_port=on  XmcBlockStatus=1  maskContainerNames=group4  block_type=gatewayin  block_config=sysgen:gateway_in_config  block_width_w=590  block_height_w=620  block_width=640  block_height=850
  slice1_x_presc_mul : hdlBasic/Gateway In  gui_display_data_type=Fixed-point  arith_type=Signed (2's comp)  n_bits=dt.const.sz  bin_pt=dt.const.bin  preci_type=Single  exp_width=8  frac_width=24  rows=1  columns=1  quantization=Truncate  overflow=Wrap  period=hw.t_axi  UseAsADC=off  ADCChannel='1'  interface=AXI4-Lite  automatic_assignment=off  address_offset=ip.offsets.slice1_cfg + hex2dec('3c')  intf_name=''  intf_description=''  default_value=0  timing_constraint=None  locs_specified=off  LOCs={}  io_standard={}  inherit_from_input=off  hdl_port=on  XmcBlockStatus=1  maskContainerNames=group4  block_type=gatewayin  block_config=sysgen:gateway_in_config  block_width_w=590  block_height_w=620  block_width=640  block_height=850
  slice1_x_presc_shift : hdlBasic/Gateway In  gui_display_data_type=Fixed-point  arith_type=Unsigned  n_bits=5  bin_pt=0  preci_type=Single  exp_width=8  frac_width=24  rows=1  columns=1  quantization=Truncate  overflow=Wrap  period=hw.t_axi  UseAsADC=off  ADCChannel='1'  interface=AXI4-Lite  automatic_assignment=off  address_offset=ip.offsets.slice1_cfg + hex2dec('38')  intf_name=''  intf_description=''  default_value=0  timing_constraint=None  locs_specified=off  LOCs={}  io_standard={}  inherit_from_input=off  hdl_port=on  XmcBlockStatus=1  maskContainerNames=group4  block_type=gatewayin  block_config=sysgen:gateway_in_config  block_width_w=590  block_height_w=620  block_width=640  block_height=850
  slice1_xd_gain : hdlBasic/Gateway In  gui_display_data_type=Fixed-point  arith_type=Signed (2's comp)  n_bits=dt.const.sz  bin_pt=dt.const.bin  preci_type=Single  exp_width=8  frac_width=24  rows=1  columns=1  quantization=Truncate  overflow=Wrap  period=hw.t_axi  UseAsADC=off  ADCChannel='1'  interface=AXI4-Lite  automatic_assignment=off  address_offset=ip.offsets.slice1_cfg + hex2dec('14')  intf_name=''  intf_description=''  default_value=0  timing_constraint=None  locs_specified=off  LOCs={}  io_standard={}  inherit_from_input=off  hdl_port=on  XmcBlockStatus=1  maskContainerNames=group4  block_type=gatewayin  block_config=sysgen:gateway_in_config  block_width_w=590  block_height_w=620  block_width=640  block_height=850
  slice1_xd_mux : hdlBasic/Gateway In  gui_display_data_type=Boolean  arith_type=Boolean  n_bits=8  bin_pt=0  preci_type=Single  exp_width=8  frac_width=24  rows=1  columns=1  quantization=Truncate  overflow=Wrap  period=hw.t_axi  UseAsADC=off  ADCChannel='1'  interface=AXI4-Lite  automatic_assignment=off  address_offset=ip.offsets.slice1_cfg + hex2dec('10')  intf_name=''  intf_description=''  default_value=0  timing_constraint=None  locs_specified=off  LOCs={}  io_standard={}  inherit_from_input=off  hdl_port=on  XmcBlockStatus=1  maskContainerNames=group4  block_type=gatewayin  block_config=sysgen:gateway_in_config  block_width_w=590  block_height_w=620  block_width=640  block_height=850
  slice1_xd_nlf_gain : hdlBasic/Gateway In  gui_display_data_type=Fixed-point  arith_type=Signed (2's comp)  n_bits=dt.const.sz  bin_pt=dt.const.bin  preci_type=Single  exp_width=8  frac_width=24  rows=1  columns=1  quantization=Truncate  overflow=Wrap  period=hw.t_axi  UseAsADC=off  ADCChannel='1'  interface=AXI4-Lite  automatic_assignment=off  address_offset=ip.offsets.slice1_cfg + hex2dec('1c')  intf_name=''  intf_description=''  default_value=0  timing_constraint=None  locs_specified=off  LOCs={}  io_standard={}  inherit_from_input=off  hdl_port=on  XmcBlockStatus=1  maskContainerNames=group4  block_type=gatewayin  block_config=sysgen:gateway_in_config  block_width_w=590  block_height_w=620  block_width=640  block_height=850
  slice1_xd_nlf_presc : hdlBasic/Gateway In  gui_display_data_type=Fixed-point  arith_type=Signed (2's comp)  n_bits=dt.const.sz  bin_pt=dt.const.bin  preci_type=Single  exp_width=8  frac_width=24  rows=1  columns=1  quantization=Truncate  overflow=Wrap  period=hw.t_axi  UseAsADC=off  ADCChannel='1'  interface=AXI4-Lite  automatic_assignment=off  address_offset=ip.offsets.slice1_cfg + hex2dec('18')  intf_name=''  intf_description=''  default_value=0  timing_constraint=None  locs_specified=off  LOCs={}  io_standard={}  inherit_from_input=off  hdl_port=on  XmcBlockStatus=1  maskContainerNames=group4  block_type=gatewayin  block_config=sysgen:gateway_in_config  block_width_w=590  block_height_w=620  block_width=640  block_height=850
  slice1_xd_presc_mul : hdlBasic/Gateway In  gui_display_data_type=Fixed-point  arith_type=Signed (2's comp)  n_bits=dt.const.sz  bin_pt=dt.const.bin  preci_type=Single  exp_width=8  frac_width=24  rows=1  columns=1  quantization=Truncate  overflow=Wrap  period=hw.t_axi  UseAsADC=off  ADCChannel='1'  interface=AXI4-Lite  automatic_assignment=off  address_offset=ip.offsets.slice1_cfg + hex2dec('34')  intf_name=''  intf_description=''  default_value=0  timing_constraint=None  locs_specified=off  LOCs={}  io_standard={}  inherit_from_input=off  hdl_port=on  XmcBlockStatus=1  maskContainerNames=group4  block_type=gatewayin  block_config=sysgen:gateway_in_config  block_width_w=590  block_height_w=620  block_width=640  block_height=850
  slice1_xd_presc_shift : hdlBasic/Gateway In  gui_display_data_type=Fixed-point  arith_type=Unsigned  n_bits=5  bin_pt=0  preci_type=Single  exp_width=8  frac_width=24  rows=1  columns=1  quantization=Truncate  overflow=Wrap  period=hw.t_axi  UseAsADC=off  ADCChannel='1'  interface=AXI4-Lite  automatic_assignment=off  address_offset=ip.offsets.slice1_cfg + hex2dec('30')  intf_name=''  intf_description=''  default_value=0  timing_constraint=None  locs_specified=off  LOCs={}  io_standard={}  inherit_from_input=off  hdl_port=on  XmcBlockStatus=1  maskContainerNames=group4  block_type=gatewayin  block_config=sysgen:gateway_in_config  block_width_w=590  block_height_w=620  block_width=640  block_height=850
  slice2_u_gain : hdlBasic/Gateway In  gui_display_data_type=Fixed-point  arith_type=Signed (2's comp)  n_bits=dt.const.sz  bin_pt=dt.const.bin  preci_type=Single  exp_width=8  frac_width=24  rows=1  columns=1  quantization=Truncate  overflow=Wrap  period=hw.t_axi  UseAsADC=off  ADCChannel='1'  interface=AXI4-Lite  automatic_assignment=off  address_offset=ip.offsets.slice2_cfg + hex2dec('24')  intf_name=''  intf_description=''  default_value=0  timing_constraint=None  locs_specified=off  LOCs={}  io_standard={}  inherit_from_input=off  hdl_port=on  XmcBlockStatus=1  maskContainerNames=group4  block_type=gatewayin  block_config=sysgen:gateway_in_config  block_width_w=590  block_height_w=620  block_width=640  block_height=850
  slice2_u_mux : hdlBasic/Gateway In  gui_display_data_type=Boolean  arith_type=Boolean  n_bits=8  bin_pt=0  preci_type=Single  exp_width=8  frac_width=24  rows=1  columns=1  quantization=Truncate  overflow=Wrap  period=hw.t_axi  UseAsADC=off  ADCChannel='1'  interface=AXI4-Lite  automatic_assignment=off  address_offset=ip.offsets.slice2_cfg + hex2dec('20')  intf_name=''  intf_description=''  default_value=0  timing_constraint=None  locs_specified=off  LOCs={}  io_standard={}  inherit_from_input=off  hdl_port=on  XmcBlockStatus=1  maskContainerNames=group4  block_type=gatewayin  block_config=sysgen:gateway_in_config  block_width_w=590  block_height_w=620  block_width=640  block_height=850
  slice2_u_nlf_gain : hdlBasic/Gateway In  gui_display_data_type=Fixed-point  arith_type=Signed (2's comp)  n_bits=dt.const.sz  bin_pt=dt.const.bin  preci_type=Single  exp_width=8  frac_width=24  rows=1  columns=1  quantization=Truncate  overflow=Wrap  period=hw.t_axi  UseAsADC=off  ADCChannel='1'  interface=AXI4-Lite  automatic_assignment=off  address_offset=ip.offsets.slice2_cfg + hex2dec('2c')  intf_name=''  intf_description=''  default_value=0  timing_constraint=None  locs_specified=off  LOCs={}  io_standard={}  inherit_from_input=off  hdl_port=on  XmcBlockStatus=1  maskContainerNames=group4  block_type=gatewayin  block_config=sysgen:gateway_in_config  block_width_w=590  block_height_w=620  block_width=640  block_height=850
  slice2_u_nlf_presc : hdlBasic/Gateway In  gui_display_data_type=Fixed-point  arith_type=Signed (2's comp)  n_bits=dt.const.sz  bin_pt=dt.const.bin  preci_type=Single  exp_width=8  frac_width=24  rows=1  columns=1  quantization=Truncate  overflow=Wrap  period=hw.t_axi  UseAsADC=off  ADCChannel='1'  interface=AXI4-Lite  automatic_assignment=off  address_offset=ip.offsets.slice2_cfg + hex2dec('28')  intf_name=''  intf_description=''  default_value=0  timing_constraint=None  locs_specified=off  LOCs={}  io_standard={}  inherit_from_input=off  hdl_port=on  XmcBlockStatus=1  maskContainerNames=group4  block_type=gatewayin  block_config=sysgen:gateway_in_config  block_width_w=590  block_height_w=620  block_width=640  block_height=850
  slice2_x_gain : hdlBasic/Gateway In  gui_display_data_type=Fixed-point  arith_type=Signed (2's comp)  n_bits=dt.const.sz  bin_pt=dt.const.bin  preci_type=Single  exp_width=8  frac_width=24  rows=1  columns=1  quantization=Truncate  overflow=Wrap  period=hw.t_axi  UseAsADC=off  ADCChannel='1'  interface=AXI4-Lite  automatic_assignment=off  address_offset=ip.offsets.slice2_cfg + hex2dec('04')  intf_name=''  intf_description=''  default_value=0  timing_constraint=None  locs_specified=off  LOCs={}  io_standard={}  inherit_from_input=off  hdl_port=on  XmcBlockStatus=1  maskContainerNames=group4  block_type=gatewayin  block_config=sysgen:gateway_in_config  block_width_w=590  block_height_w=620  block_width=640  block_height=850
  slice2_x_mux : hdlBasic/Gateway In  gui_display_data_type=Boolean  arith_type=Boolean  n_bits=8  bin_pt=0  preci_type=Single  exp_width=8  frac_width=24  rows=1  columns=1  quantization=Truncate  overflow=Wrap  period=hw.t_axi  UseAsADC=off  ADCChannel='1'  interface=AXI4-Lite  automatic_assignment=off  address_offset=ip.offsets.slice2_cfg + hex2dec('00')  intf_name=''  intf_description=''  default_value=0  timing_constraint=None  locs_specified=off  LOCs={}  io_standard={}  inherit_from_input=off  hdl_port=on  XmcBlockStatus=1  maskContainerNames=group4  block_type=gatewayin  block_config=sysgen:gateway_in_config  block_width_w=590  block_height_w=620  block_width=640  block_height=850
  slice2_x_nlf_gain : hdlBasic/Gateway In  gui_display_data_type=Fixed-point  arith_type=Signed (2's comp)  n_bits=dt.const.sz  bin_pt=dt.const.bin  preci_type=Single  exp_width=8  frac_width=24  rows=1  columns=1  quantization=Truncate  overflow=Wrap  period=hw.t_axi  UseAsADC=off  ADCChannel='1'  interface=AXI4-Lite  automatic_assignment=off  address_offset=ip.offsets.slice2_cfg + hex2dec('0c')  intf_name=''  intf_description=''  default_value=0  timing_constraint=None  locs_specified=off  LOCs={}  io_standard={}  inherit_from_input=off  hdl_port=on  XmcBlockStatus=1  maskContainerNames=group4  block_type=gatewayin  block_config=sysgen:gateway_in_config  block_width_w=590  block_height_w=620  block_width=640  block_height=850
  slice2_x_nlf_presc : hdlBasic/Gateway In  gui_display_data_type=Fixed-point  arith_type=Signed (2's comp)  n_bits=dt.const.sz  bin_pt=dt.const.bin  preci_type=Single  exp_width=8  frac_width=24  rows=1  columns=1  quantization=Truncate  overflow=Wrap  period=hw.t_axi  UseAsADC=off  ADCChannel='1'  interface=AXI4-Lite  automatic_assignment=off  address_offset=ip.offsets.slice2_cfg + hex2dec('08')  intf_name=''  intf_description=''  default_value=0  timing_constraint=None  locs_specified=off  LOCs={}  io_standard={}  inherit_from_input=off  hdl_port=on  XmcBlockStatus=1  maskContainerNames=group4  block_type=gatewayin  block_config=sysgen:gateway_in_config  block_width_w=590  block_height_w=620  block_width=640  block_height=850
  slice2_x_presc_mul : hdlBasic/Gateway In  gui_display_data_type=Fixed-point  arith_type=Signed (2's comp)  n_bits=dt.const.sz  bin_pt=dt.const.bin  preci_type=Single  exp_width=8  frac_width=24  rows=1  columns=1  quantization=Truncate  overflow=Wrap  period=hw.t_axi  UseAsADC=off  ADCChannel='1'  interface=AXI4-Lite  automatic_assignment=off  address_offset=ip.offsets.slice2_cfg + hex2dec('3c')  intf_name=''  intf_description=''  default_value=0  timing_constraint=None  locs_specified=off  LOCs={}  io_standard={}  inherit_from_input=off  hdl_port=on  XmcBlockStatus=1  maskContainerNames=group4  block_type=gatewayin  block_config=sysgen:gateway_in_config  block_width_w=590  block_height_w=620  block_width=640  block_height=850
  slice2_x_presc_shift : hdlBasic/Gateway In  gui_display_data_type=Fixed-point  arith_type=Unsigned  n_bits=5  bin_pt=0  preci_type=Single  exp_width=8  frac_width=24  rows=1  columns=1  quantization=Truncate  overflow=Wrap  period=hw.t_axi  UseAsADC=off  ADCChannel='1'  interface=AXI4-Lite  automatic_assignment=off  address_offset=ip.offsets.slice2_cfg + hex2dec('38')  intf_name=''  intf_description=''  default_value=0  timing_constraint=None  locs_specified=off  LOCs={}  io_standard={}  inherit_from_input=off  hdl_port=on  XmcBlockStatus=1  maskContainerNames=group4  block_type=gatewayin  block_config=sysgen:gateway_in_config  block_width_w=590  block_height_w=620  block_width=640  block_height=850
  slice2_xd_gain : hdlBasic/Gateway In  gui_display_data_type=Fixed-point  arith_type=Signed (2's comp)  n_bits=dt.const.sz  bin_pt=dt.const.bin  preci_type=Single  exp_width=8  frac_width=24  rows=1  columns=1  quantization=Truncate  overflow=Wrap  period=hw.t_axi  UseAsADC=off  ADCChannel='1'  interface=AXI4-Lite  automatic_assignment=off  address_offset=ip.offsets.slice2_cfg + hex2dec('14')  intf_name=''  intf_description=''  default_value=0  timing_constraint=None  locs_specified=off  LOCs={}  io_standard={}  inherit_from_input=off  hdl_port=on  XmcBlockStatus=1  maskContainerNames=group4  block_type=gatewayin  block_config=sysgen:gateway_in_config  block_width_w=590  block_height_w=620  block_width=640  block_height=850
  slice2_xd_mux : hdlBasic/Gateway In  gui_display_data_type=Boolean  arith_type=Boolean  n_bits=8  bin_pt=0  preci_type=Single  exp_width=8  frac_width=24  rows=1  columns=1  quantization=Truncate  overflow=Wrap  period=hw.t_axi  UseAsADC=off  ADCChannel='1'  interface=AXI4-Lite  automatic_assignment=off  address_offset=ip.offsets.slice2_cfg + hex2dec('10')  intf_name=''  intf_description=''  default_value=0  timing_constraint=None  locs_specified=off  LOCs={}  io_standard={}  inherit_from_input=off  hdl_port=on  XmcBlockStatus=1  maskContainerNames=group4  block_type=gatewayin  block_config=sysgen:gateway_in_config  block_width_w=590  block_height_w=620  block_width=640  block_height=850
  slice2_xd_nlf_gain : hdlBasic/Gateway In  gui_display_data_type=Fixed-point  arith_type=Signed (2's comp)  n_bits=dt.const.sz  bin_pt=dt.const.bin  preci_type=Single  exp_width=8  frac_width=24  rows=1  columns=1  quantization=Truncate  overflow=Wrap  period=hw.t_axi  UseAsADC=off  ADCChannel='1'  interface=AXI4-Lite  automatic_assignment=off  address_offset=ip.offsets.slice2_cfg + hex2dec('1c')  intf_name=''  intf_description=''  default_value=0  timing_constraint=None  locs_specified=off  LOCs={}  io_standard={}  inherit_from_input=off  hdl_port=on  XmcBlockStatus=1  maskContainerNames=group4  block_type=gatewayin  block_config=sysgen:gateway_in_config  block_width_w=590  block_height_w=620  block_width=640  block_height=850
  slice2_xd_nlf_presc : hdlBasic/Gateway In  gui_display_data_type=Fixed-point  arith_type=Signed (2's comp)  n_bits=dt.const.sz  bin_pt=dt.const.bin  preci_type=Single  exp_width=8  frac_width=24  rows=1  columns=1  quantization=Truncate  overflow=Wrap  period=hw.t_axi  UseAsADC=off  ADCChannel='1'  interface=AXI4-Lite  automatic_assignment=off  address_offset=ip.offsets.slice2_cfg + hex2dec('18')  intf_name=''  intf_description=''  default_value=0  timing_constraint=None  locs_specified=off  LOCs={}  io_standard={}  inherit_from_input=off  hdl_port=on  XmcBlockStatus=1  maskContainerNames=group4  block_type=gatewayin  block_config=sysgen:gateway_in_config  block_width_w=590  block_height_w=620  block_width=640  block_height=850
  slice2_xd_presc_mul : hdlBasic/Gateway In  gui_display_data_type=Fixed-point  arith_type=Signed (2's comp)  n_bits=dt.const.sz  bin_pt=dt.const.bin  preci_type=Single  exp_width=8  frac_width=24  rows=1  columns=1  quantization=Truncate  overflow=Wrap  period=hw.t_axi  UseAsADC=off  ADCChannel='1'  interface=AXI4-Lite  automatic_assignment=off  address_offset=ip.offsets.slice2_cfg + hex2dec('34')  intf_name=''  intf_description=''  default_value=0  timing_constraint=None  locs_specified=off  LOCs={}  io_standard={}  inherit_from_input=off  hdl_port=on  XmcBlockStatus=1  maskContainerNames=group4  block_type=gatewayin  block_config=sysgen:gateway_in_config  block_width_w=590  block_height_w=620  block_width=640  block_height=850
  slice2_xd_presc_shift : hdlBasic/Gateway In  gui_display_data_type=Fixed-point  arith_type=Unsigned  n_bits=5  bin_pt=0  preci_type=Single  exp_width=8  frac_width=24  rows=1  columns=1  quantization=Truncate  overflow=Wrap  period=hw.t_axi  UseAsADC=off  ADCChannel='1'  interface=AXI4-Lite  automatic_assignment=off  address_offset=ip.offsets.slice2_cfg + hex2dec('30')  intf_name=''  intf_description=''  default_value=0  timing_constraint=None  locs_specified=off  LOCs={}  io_standard={}  inherit_from_input=off  hdl_port=on  XmcBlockStatus=1  maskContainerNames=group4  block_type=gatewayin  block_config=sysgen:gateway_in_config  block_width_w=590  block_height_w=620  block_width=640  block_height=850
  system_run : hdlBasic/Gateway In  gui_display_data_type=Boolean  arith_type=Boolean  n_bits=32  bin_pt=0  preci_type=Single  exp_width=8  frac_width=24  rows=1  columns=1  quantization=Truncate  overflow=Wrap  period=hw.t_axi  UseAsADC=off  ADCChannel='1'  interface=AXI4-Lite  automatic_assignment=off  address_offset=ip.offsets.system_cfg + hex2dec('00')  intf_name=''  intf_description=''  default_value=0  timing_constraint=None  locs_specified=off  LOCs={}  io_standard={}  inherit_from_input=off  hdl_port=on  XmcBlockStatus=1  maskContainerNames=group4  block_type=gatewayin  block_config=sysgen:gateway_in_config  block_width_w=590  block_height_w=620  block_width=640  block_height=850
  axiclk_system_reset : Outport
  axiclk_system_run : Outport  Port=2
  axiclk_led : Outport  Port=3
  axiclk_cfg_nlf_addr : Outport  Port=4
  axiclk_cfg_nlf_data : Outport  Port=5
  axiclk_cfg_nlf_we : Outport  Port=6
  axiclk_cfg_nlf_start : Outport  Port=7
  axiclk_noise0_presc : Outport  Port=8
  axiclk_noise1_presc : Outport  Port=9
  axiclk_noise2_presc : Outport  Port=10
  axiclk_nlf_cfg_select : Outport  Port=11
  axiclk_input_matrix_cfg : Outport  Port=12
  axiclk_output_matrix_cfg : Outport  Port=13
  axiclk_slice0_cfg : Outport  Port=14
  axiclk_slice1_cfg : Outport  Port=15
  axiclk_slice2_cfg : Outport  Port=16
  axiclk_adc_nlf_cfg : Outport  Port=17
  axiclk_adc_calib_in : Outport  Port=18
  axiclk_dac_calib : Outport  Port=19
  axiclk_nlf_sw_io_mask : Outport  Port=20
  axiclk_nlf_sw_software_sel : Outport  Port=21
  wires:
  led_value/1 -> axiclk_led/1
  slice1_x_mux/1 -> Bus Creator/1
  slice1_x_gain/1 -> Bus Creator/2
  slice1_x_nlf_presc/1 -> Bus Creator/3
  slice1_x_nlf_gain/1 -> Bus Creator/4
  Constant/1 -> slice1_x_mux/1
  Constant1/1 -> slice1_x_gain/1
  Constant3/1 -> slice1_x_nlf_gain/1
  Constant2/1 -> slice1_x_nlf_presc/1
  slice1_xd_mux/1 -> Bus Creator/5
  slice1_xd_gain/1 -> Bus Creator/6
  slice1_xd_nlf_presc/1 -> Bus Creator/7
  slice1_xd_nlf_gain/1 -> Bus Creator/8
  Constant8/1 -> slice1_xd_mux/1
  Constant9/1 -> slice1_xd_gain/1
  Constant10/1 -> slice1_xd_nlf_presc/1
  Constant11/1 -> slice1_xd_nlf_gain/1
  slice1_u_mux/1 -> Bus Creator/9
  slice1_u_gain/1 -> Bus Creator/10
  slice1_u_nlf_presc/1 -> Bus Creator/11
  slice1_u_nlf_gain/1 -> Bus Creator/12
  Constant14/1 -> slice1_u_mux/1
  Constant15/1 -> slice1_u_gain/1
  Constant12/1 -> slice1_u_nlf_presc/1
  Constant13/1 -> slice1_u_nlf_gain/1
  Constant16/1 -> led_value/1
  cfg_nlf_select/1 -> cfg_nlf_select[7:0]/1
  Constant17/1 -> cfg_nlf_select/1
  cfg_nlf_addr/1 -> axiclk_cfg_nlf_addr/1
  cfg_nlf_data/1 -> axiclk_cfg_nlf_data/1
  cfg_nlf_we/1 -> axiclk_cfg_nlf_we/1
  cfg_nlf_start/1 -> axiclk_cfg_nlf_start/1
  axiclk_cfg_nlf_done/1 -> cfg_nlf_done/1
  Constant18/1 -> cfg_nlf_addr/1
  Constant19/1 -> cfg_nlf_data/1
  Constant20/1 -> cfg_nlf_we/1
  Constant21/1 -> cfg_nlf_start/1
  cfg_nlf_done/1 -> Terminator/1
  Constant22/1 -> system_run/1
  system_run/1 -> axiclk_system_run/1
  Constant26/1 -> slice1_xd_presc_mul/1
  Constant23/1 -> slice1_x_presc_shift/1
  Constant24/1 -> slice1_x_presc_mul/1
  Constant25/1 -> slice1_xd_presc_shift/1
  slice1_xd_presc_shift/1 -> Bus Creator/13
  slice1_xd_presc_mul/1 -> Bus Creator/14
  slice1_x_presc_shift/1 -> Bus Creator/15
  slice1_x_presc_mul/1 -> Bus Creator/16
  inp_mat_fac_u0_adc0/1 -> Bus Creator2/1
  inp_mat_fac_u0_adc1/1 -> Bus Creator2/2
  inp_mat_fac_u0_noise/1 -> Bus Creator2/3
  inp_mat_fac_u1_adc0/1 -> Bus Creator2/4
  inp_mat_fac_u1_adc1/1 -> Bus Creator2/5
  inp_mat_fac_u1_noise/1 -> Bus Creator2/6
  inp_mat_fac_u2_adc0/1 -> Bus Creator2/7
  inp_mat_fac_u2_adc1/1 -> Bus Creator2/8
  inp_mat_fac_u2_noise/1 -> Bus Creator2/9
  Bus Creator2/1 -> axiclk_input_matrix_cfg/1
  Constant27/1 -> inp_mat_fac_u0_adc0/1
  Constant28/1 -> inp_mat_fac_u0_adc1/1
  Constant29/1 -> inp_mat_fac_u0_noise/1
  Constant30/1 -> inp_mat_fac_u1_adc0/1
  Constant31/1 -> inp_mat_fac_u1_adc1/1
  Constant32/1 -> inp_mat_fac_u1_noise/1
  Constant33/1 -> inp_mat_fac_u2_adc0/1
  Constant34/1 -> inp_mat_fac_u2_adc1/1
  Constant35/1 -> inp_mat_fac_u2_noise/1
  out_mat_dac0_selx0/1 -> Bus Creator3/1
  out_mat_dac0_selx1/1 -> Bus Creator3/2
  out_mat_dac0_selx2/1 -> Bus Creator3/3
  out_mat_fac_dac0_xx0/1 -> Bus Creator3/4
  out_mat_fac_dac0_xx1/1 -> Bus Creator3/5
  out_mat_fac_dac0_xx2/1 -> Bus Creator3/6
  out_mat_dac1_selx0/1 -> Bus Creator3/7
  out_mat_dac1_selx1/1 -> Bus Creator3/8
  out_mat_dac1_selx2/1 -> Bus Creator3/9
  out_mat_fac_dac1_xx0/1 -> Bus Creator3/10
  out_mat_fac_dac1_xx1/1 -> Bus Creator3/11
  out_mat_fac_dac1_xx2/1 -> Bus Creator3/12
  Bus Creator3/1 -> axiclk_output_matrix_cfg/1
  Constant39/1 -> out_mat_dac0_selx0/1
  Constant41/1 -> out_mat_dac0_selx2/1
  Constant40/1 -> out_mat_dac0_selx1/1
  Constant42/1 -> out_mat_dac1_selx0/1
  Constant43/1 -> out_mat_dac1_selx1/1
  Constant44/1 -> out_mat_dac1_selx2/1
  Constant45/1 -> out_mat_fac_dac0_xx0/1
  Constant46/1 -> out_mat_fac_dac0_xx1/1
  Constant47/1 -> out_mat_fac_dac0_xx2/1
  Constant48/1 -> out_mat_fac_dac1_xx0/1
  Constant49/1 -> out_mat_fac_dac1_xx1/1
  Constant50/1 -> out_mat_fac_dac1_xx2/1
  Bus Creator/1 -> axiclk_slice1_cfg/1
  Constant60/1 -> slice0_x_presc_shift/1
  slice0_x_nlf_presc/1 -> Bus Creator4/3
  Constant61/1 -> slice0_x_presc_mul/1
  Constant53/1 -> slice0_xd_nlf_presc/1
  slice0_xd_presc_mul/1 -> Bus Creator4/14
  slice0_u_gain/1 -> Bus Creator4/10
  slice0_x_presc_shift/1 -> Bus Creator4/15
  Constant52/1 -> slice0_x_gain/1
  slice0_x_mux/1 -> Bus Creator4/1
  Constant56/1 -> slice0_u_nlf_gain/1
  Constant66/1 -> slice0_xd_gain/1
  slice0_xd_nlf_presc/1 -> Bus Creator4/7
  slice0_x_nlf_gain/1 -> Bus Creator4/4
  slice0_u_mux/1 -> Bus Creator4/9
  slice0_xd_mux/1 -> Bus Creator4/5
  Constant64/1 -> slice0_x_nlf_gain/1
  Constant51/1 -> slice0_x_mux/1
  Constant62/1 -> slice0_xd_presc_shift/1
  Constant54/1 -> slice0_xd_nlf_gain/1
  slice0_xd_gain/1 -> Bus Creator4/6
  Constant65/1 -> slice0_xd_mux/1
  slice0_x_gain/1 -> Bus Creator4/2
  slice0_u_nlf_gain/1 -> Bus Creator4/12
  Bus Creator4/1 -> axiclk_slice0_cfg/1
  Constant58/1 -> slice0_u_gain/1
  Constant55/1 -> slice0_u_nlf_presc/1
  Constant57/1 -> slice0_u_mux/1
  slice0_xd_nlf_gain/1 -> Bus Creator4/8
  Constant63/1 -> slice0_xd_presc_mul/1
  Constant59/1 -> slice0_x_nlf_presc/1
  slice0_u_nlf_presc/1 -> Bus Creator4/11
  slice0_x_presc_mul/1 -> Bus Creator4/16
  slice0_xd_presc_shift/1 -> Bus Creator4/13
  Constant76/1 -> slice2_x_presc_shift/1
  slice2_x_nlf_presc/1 -> Bus Creator5/3
  Constant77/1 -> slice2_x_presc_mul/1
  Constant69/1 -> slice2_xd_nlf_presc/1
  slice2_xd_presc_mul/1 -> Bus Creator5/14
  slice2_u_gain/1 -> Bus Creator5/10
  slice2_x_presc_shift/1 -> Bus Creator5/15
  Constant68/1 -> slice2_x_gain/1
  slice2_x_mux/1 -> Bus Creator5/1
  Constant72/1 -> slice2_u_nlf_gain/1
  Constant82/1 -> slice2_xd_gain/1
  slice2_xd_nlf_presc/1 -> Bus Creator5/7
  slice2_x_nlf_gain/1 -> Bus Creator5/4
  slice2_u_mux/1 -> Bus Creator5/9
  slice2_xd_mux/1 -> Bus Creator5/5
  Constant80/1 -> slice2_x_nlf_gain/1
  Constant67/1 -> slice2_x_mux/1
  Constant78/1 -> slice2_xd_presc_shift/1
  Constant70/1 -> slice2_xd_nlf_gain/1
  slice2_xd_gain/1 -> Bus Creator5/6
  Constant81/1 -> slice2_xd_mux/1
  slice2_x_gain/1 -> Bus Creator5/2
  slice2_u_nlf_gain/1 -> Bus Creator5/12
  Bus Creator5/1 -> axiclk_slice2_cfg/1
  Constant74/1 -> slice2_u_gain/1
  Constant71/1 -> slice2_u_nlf_presc/1
  Constant73/1 -> slice2_u_mux/1
  slice2_xd_nlf_gain/1 -> Bus Creator5/8
  Constant79/1 -> slice2_xd_presc_mul/1
  Constant75/1 -> slice2_x_nlf_presc/1
  slice2_u_nlf_presc/1 -> Bus Creator5/11
  slice2_x_presc_mul/1 -> Bus Creator5/16
  slice2_xd_presc_shift/1 -> Bus Creator5/13
  cfg_noise_presc0/1 -> axiclk_noise0_presc/1
  cfg_noise_presc1/1 -> axiclk_noise1_presc/1
  cfg_noise_presc2/1 -> axiclk_noise2_presc/1
  Constant83/1 -> cfg_noise_presc0/1
  Constant84/1 -> cfg_noise_presc1/1
  Constant85/1 -> cfg_noise_presc2/1
  Bus Creator6/1 -> axiclk_adc_nlf_cfg/1
  adc0_nlf_presc/1 -> Bus Creator6/1
  adc0_nlf_gain/1 -> Bus Creator6/2
  adc0_nlf_enable/1 -> Bus Creator6/3
  adc1_nlf_presc/1 -> Bus Creator6/4
  adc1_nlf_gain/1 -> Bus Creator6/5
  adc1_nlf_enable/1 -> Bus Creator6/6
  Constant4/1 -> adc0_nlf_presc/1
  Constant5/1 -> adc0_nlf_gain/1
  Constant7/1 -> adc0_nlf_enable/1
  Constant6/1 -> adc1_nlf_presc/1
  Constant86/1 -> adc1_nlf_gain/1
  Constant87/1 -> adc1_nlf_enable/1
  Constant94/1 -> cfg_system_reset/1
  cfg_system_reset/1 -> axiclk_system_reset/1
  adc0_calib_offset/1 -> Bus Creator8/1
  adc1_calib_offset/1 -> Bus Creator8/2
  Bus Selector/1 -> adc0_value/1  "<signal1>"
  Bus Selector/2 -> adc1_value/1  "<signal2>"
  Constant95/1 -> adc0_calib_offset/1
  Constant96/1 -> adc1_calib_offset/1
  adc0_value/1 -> Terminator1/1
  adc1_value/1 -> Terminator2/1
  Bus Creator8/1 -> axiclk_adc_calib_in/1
  axiclk_adc_calib_out/1 -> Bus Selector/1
  adc0_calib_factor/1 -> Bus Creator8/3
  adc1_calib_factor/1 -> Bus Creator8/4
  Constant97/1 -> adc0_calib_factor/1
  Constant98/1 -> adc1_calib_factor/1
  Constant36/1 -> out_mat_nlf_dac0_xx0_en/1
  Constant37/1 -> out_mat_nlf_dac0_xx0_presc/1
  Constant38/1 -> out_mat_nlf_dac0_xx0_gain/1
  Constant88/1 -> out_mat_nlf_dac0_xx1_en/1
  Constant90/1 -> out_mat_nlf_dac0_xx1_gain/1
  Constant89/1 -> out_mat_nlf_dac0_xx1_presc/1
  Constant92/1 -> out_mat_nlf_dac0_xx2_presc/1
  Constant91/1 -> out_mat_nlf_dac0_xx2_en/1
  Constant93/1 -> out_mat_nlf_dac0_xx2_gain/1
  Constant107/1 -> out_mat_nlf_dac1_xx2_gain/1
  Constant103/1 -> out_mat_nlf_dac1_xx1_presc/1
  Constant101/1 -> out_mat_nlf_dac1_xx0_gain/1
  Constant105/1 -> out_mat_nlf_dac1_xx2_en/1
  Constant102/1 -> out_mat_nlf_dac1_xx1_en/1
  Constant106/1 -> out_mat_nlf_dac1_xx2_presc/1
  Constant99/1 -> out_mat_nlf_dac1_xx0_en/1
  Constant104/1 -> out_mat_nlf_dac1_xx1_gain/1
  Constant100/1 -> out_mat_nlf_dac1_xx0_presc/1
  out_mat_nlf_dac0_xx0_en/1 -> Bus Creator3/13
  out_mat_nlf_dac0_xx0_presc/1 -> Bus Creator3/14
  out_mat_nlf_dac0_xx0_gain/1 -> Bus Creator3/15
  out_mat_nlf_dac0_xx1_en/1 -> Bus Creator3/16
  out_mat_nlf_dac0_xx1_presc/1 -> Bus Creator3/17
  out_mat_nlf_dac0_xx1_gain/1 -> Bus Creator3/18
  out_mat_nlf_dac0_xx2_en/1 -> Bus Creator3/19
  out_mat_nlf_dac0_xx2_presc/1 -> Bus Creator3/20
  out_mat_nlf_dac0_xx2_gain/1 -> Bus Creator3/21
  out_mat_nlf_dac1_xx0_en/1 -> Bus Creator3/22
  out_mat_nlf_dac1_xx0_presc/1 -> Bus Creator3/23
  out_mat_nlf_dac1_xx0_gain/1 -> Bus Creator3/24
  out_mat_nlf_dac1_xx1_en/1 -> Bus Creator3/25
  out_mat_nlf_dac1_xx1_presc/1 -> Bus Creator3/26
  out_mat_nlf_dac1_xx1_gain/1 -> Bus Creator3/27
  out_mat_nlf_dac1_xx2_en/1 -> Bus Creator3/28
  out_mat_nlf_dac1_xx2_presc/1 -> Bus Creator3/29
  out_mat_nlf_dac1_xx2_gain/1 -> Bus Creator3/30
  Constant108/1 -> dac0_calib_offset/1
  Constant109/1 -> dac1_calib_offset/1
  Constant110/1 -> dac0_calib_factor/1
  Constant111/1 -> dac1_calib_factor/1
  dac0_calib_offset/1 -> Bus Creator7/1
  dac1_calib_offset/1 -> Bus Creator7/2
  dac0_calib_factor/1 -> Bus Creator7/3
  dac1_calib_factor/1 -> Bus Creator7/4
  Bus Creator7/1 -> axiclk_dac_calib/1
  cfg_nlf_select[7:0]/1 -> axiclk_nlf_cfg_select/1
  axiclk_nlf_switch/1 -> nlf_switch/1
  nlf_switch/1 -> Terminator3/1
  Constant112/1 -> nlf_switch_io_mask/1
  Constant113/1 -> nlf_switch_sw_switch/1
  nlf_switch_io_mask/1 -> axiclk_nlf_sw_io_mask/1
  nlf_switch_sw_switch/1 -> axiclk_nlf_sw_software_sel/1
